simulink library "allblocks_alteradspbuilder2"  (Simulink 7.6)
settings: Solver=ode45  StartTime=0.0  StopTime=10.0  RelTol=1e-3
InitFcn:
  | %% DSPBuilder Start
  | alt_dspbuilder_update_model(bdroot)
  | %% DSPBuilder End
undefined symbols (not defined in the file): alt_dspbuilder_internal_AvalonSTPFC_generate, alt_dspbuilder_internal_init_altlab_flow, alt_dspbuilder_internal_init_blackbox_flow, alt_dspbuilder_internal_initfcn_base_clock, alt_dspbuilder_internal_initfcn_clock, alt_dspbuilder_internal_initfcn_pll, alt_dspbuilder_load_block, alt_dspbuilder_update_external_RAM, Inferred
libraries: allblocks_alteradspbuilder2 x15
(part 1 of 4)
settings Model: ForwardingTableString=||__slOldName__||allblocks_alteradspbuilder2/Stratix III DSP Block||__slNewName__||allblocks_alteradspbuilder2/DSP Block  Creator=swbuild  LastModifiedBy=swbuild

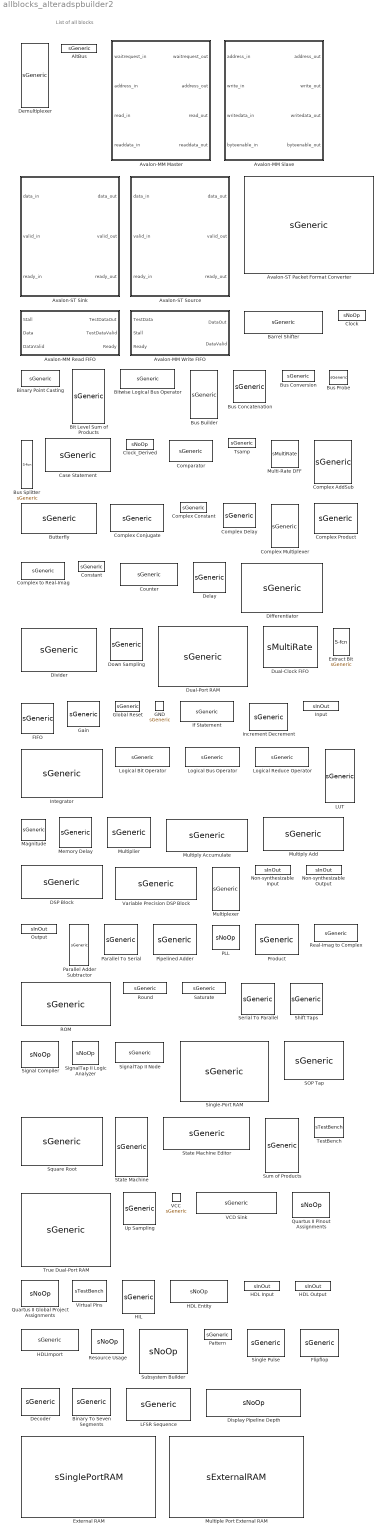
== system allblocks_alteradspbuilder2 ==
  note: List of all blocks
  AltBus : S-Function  LoadFcn=alt_dspbuilder_load_block(gcb, 'BlockFactory', 'com.altera.dspbuilder.blockset.iobus.AltBus');  FunctionName=sGeneric  Parameters=BusType bwl bwr saturate floatingPointInput floatingPointOutput logOutputs logFile  EnableBusSupport=off  mask(AltBus AlteraBlockset){BusType=Signed Integer, bwl=8, bwr=0, saturate=off, floatingPointInput=on, floatingPointOutput=on, logOutputs=off, logFile=D:\\allblocks%5Falteradspbuilder2_AltBus.fixedpointlog}
      mask prompts: BusType "Bus Type"; bwl "[Number Of Bits].[]"; bwr "[].[Number Of Bits]"; saturate "Saturate Output"; floatingPointInput "Allow Floating Point Input For This Block"; floatingPointOutput "Allow Floating Point Output For This Block"
      mask help:
      | Modifies the bus format of a DSP Builder signal. This block can only be used as an internal node in a system, not as an input to or output from the system. If the specified bit width is wider than the input bit width, the bus is sign extended to fit. If it is smaller than the input bit width, you can choose to either truncate or saturate the excess bits
      |
      | If the signal feeding the block has a different format, it is automatically cast to the type specified by the block, and Signal Compiler automatically inserts the hardware cast (if necessary).
      mask init:
      | alt_dspbuilder_init('BlockFactory', 'com.altera.dspbuilder.blockset.iobus.AltBus', { get_param(gcb, 'BusType') bwl bwr saturate floatingPointInput floatingPointOutput logOutputs logFile });
      settings: CopyFcn=alt_dspbuilder_add_block(gcb, 'BlockFactory', 'com.altera.dspbuilder.blockset.iobus.AltBus');  DeleteFcn=com.altera.dspbuilder.simulation.Mask.delete(gcb);  UndoDeleteFcn=alt_dspbuilder_add_block(gcb, 'BlockFactory', 'com.altera.dspbuilder.blockset.iobus.AltBus');  PostSaveFcn=alt_dspbuilder_block_saved(gcb);  NameChangeFcn=alt_dspbuilder_block_renamed(gcb);
      mask Help: helpview(char(com.altera.dspbuilder.simulation.Cache.getBlockTemplate('BlockFactory', 'com.altera.dspbuilder.blockset.iobus.AltBus').getHelpFile))
      mask StyleString: popup(Signed Integer|Unsigned Integer|Signed Fractional|Unsigned Fractional|Single Bit),edit,edit,checkbox,checkbox,checkbox,checkbox,edit
      mask CallbackString: alt_dspbuilder_update_gui('BlockFactory', 'com.altera.dspbuilder.blockset.iobus.AltBus', 'BusType', 0);|||||||
      mask Display:
      | plot([0 0.2 0 1 0.8 1 0], [0 0.5 1 1 0.5 0 0])
      | plot([0.08 0.28 0.08 0.92 0.72 0.92 0.08], [0 0.5 1 1 0.5 0 0])
      | disp('7:0')
  Avalon-MM Master : Subsystem  mask(Avalon-MM Master AlteraBlockset){iofile=D:\\allblocks%5Falteradspbuilder2_Avalon-MM+Master_waitrequest.salt,D:\\allblocks%5Falteradspbuilder2_Avalon-MM+Master_address.capture,D:\\allblocks%5Falteradspbuilder2_Avalon-MM+Master_read.capture,D:\\allblocks%5Falteradspbuilder2_Avalon-MM+Master_readdata.salt,, SpecifyClock=off, clock=, addrWidth=2, addrType=Read, BusType=Signed Integer, bwl=8, bwr=0, byteEnable=off, flowCtrl=off, pipeline=off, flush=off, burst=off, maxBurst=4, irq=off, irq_mode=Prioritized, externalType=Inferred, PORTTYPE=Input}
      mask prompts: SpecifyClock "Specify Clock"; addrWidth "Address Width"; addrType "Address Type"; BusType "DataType"; bwl "[number of bits].[]"; bwr "[].[number of bits]"; byteEnable "Allow Byte Enable"; flowCtrl "Allow Flow Control"; pipeline "Allow Pipeline Transfers"; flush "Use Flush Signal"; burst "Allow Burst Transfers"; maxBurst "Maximum Burst Size"; irq "Receive IRQ"; irq_mode "IRQ Mode"; externalType "External Type"; PORTTYPE "TYPE"
      mask help: Defines a collection of ports for connection to an SOPC Builder system when your design functions as an Avalon Memory-Mapped master interface.
      mask init:
      | alt_dspbuilder_internal_initBusIOBlock('BlockFactory', 'com.altera.dspbuilder.blockset.avalonmm.Master', { iofile get_param(gcb, 'SpecifyClock') clock addrWidth get_param(gcb, 'addrType') get_param(gcb, 'BusType') bwl bwr byteEnable get_param(gcb, 'flowCtrl') get_param(gcb, 'pipeline') get_param(gcb, 'flush') get_param(gcb, 'burst') maxBurst get_param(gcb, 'irq') get_param(gcb, 'irq_mode') externalType PORTTYPE });
      mask Help: helpview(char(com.altera.dspbuilder.simulation.Cache.getBlockTemplate('BlockFactory', 'com.altera.dspbuilder.blockset.avalonmm.Master').getHelpFile))
      mask StyleString: edit,checkbox,edit,edit,popup(Read|Write|Read/Write),popup(Signed Integer|Unsigned Integer|Signed Fractional|Unsigned Fractional),edit,edit,checkbox,checkbox,checkbox,checkbox,checkbox,edit,checkbox,popup(Prioritized|Indiviual Signals),popup(Inferred|Simulink Fixed Point Type|Double),edit
      mask CallbackString: |alt_dspbuilder_update_gui('BlockFactory', 'com.altera.dspbuilder.blockset.avalonmm.Master', 'SpecifyClock', 1);|||alt_dspbuilder_update_gui('BlockFactory', 'com.altera.dspbuilder.blockset.avalonmm.Master', 'addrType', 4);|alt_dspbuilder_update_gui('BlockFactory', 'com.altera.dspbuilder.blockset.avalonmm.Master', 'BusType', 5);||||alt_dspbuilder_update_gui('BlockFactory', 'com.altera.dspbuilder.blockset.avalonmm.Master', 'flowCtrl', 9);|alt_dspbuilder_update_gui('BlockFactory', 'com.altera.dspbuilder.blockset.avalonmm.Master', 'pipeline', 10);|alt_dspbuilder_update_gui('BlockFactory', 'com.altera.dspbuilder.blockset.avalonmm.Master', 'flush', 11);|alt_dspbuilder_update_gui('BlockFactory', 'com.altera.dspbuilder.blockset.avalonmm.Master', 'burst', 12);||alt_dspbuilder_update_gui('BlockFactory', 'com.altera.dspbuilder.blockset.avalonmm.Master', 'irq', 14);|alt_dspbuilder_update_gui('BlockFactory', 'com.altera.dspbuilder.blockset.avalonmm.Master', 'irq_mode', 15);||
      mask Display:
      | plot([-25 15 25 15 -25 -25]*1, [0 0 -10 -20 -20 0] - 0);
      | text(0, -10, 'Wait Request\nibit', 'horizontalAlignment','center','verticalAlignment','middle');
      | plot([-25 15 25 15 -25 -25]*-1, [0 0 -10 -20 -20 0] - 21);
      | plot([11 21 11]*-1, [0 -10 -20] - 21);
      | text(0, -31, 'Address\no1:0', 'horizontalAlignment','center','verticalAlignment','middle');
      | plot([-25 15 25 15 -25 -25]*-1, [0 0 -10 -20 -20 0] - 42);
      | text(0, -52, 'Read\nobit', 'horizontalAlignment','center','verticalAlignment','middle');
      | plot([-25 15 25 15 -25 -25]*1, [0 0 -10 -20 -20 0] - 63);
      | plot([11 21 11]*1, [0 -10 -20] - 63);
      | text(0, -73, 'Read Data\ni7:0', 'horizontalAlignment','center','verticalAlignment','middle');
  Avalon-MM Read FIFO : Subsystem  mask(Avalon-MM Read FIFO AlteraBlockSet){sgn=Signed Integer, bwl=8, bwr=3, depth=11, burst=0}
      mask prompts: sgn "Data Type"; bwl "[number of bits].[]"; bwr "[].[number of bits]"; depth "FIFO Depth"; burst "Max Burst"
      mask help:
      | Avalon-MM Read FIFO
      |
      | Implements a FIFO with Avalon-MM connectivity. Accessed by other Avalon-MM peripherals to obtain datawhen connected in SOPC Builder.
      |
      | Inputs:
      | Stall - Connect to Simulink blocks.
      | 	Used to simulate stall conditions of the Avalon-MM bus.
      | Data - Connect to DSP Builder blocks.
      | 	Used to collect outgoing data from the user design.
      | DataValid - Connect to DSP Builder blocks.
      | 	Should be asserted whenever the signal on the Data port corresponds to real data.
      |
      | Outputs:
      | TestDataOut - Connect to Simulink blocks.
      | 	Corresponds to the data received over the Avalon-MM bus.
      | TestDataValid - Connect to Simulink blocks.
      | 	Asserted whenever TestDataOut corresponds to real data.
      | Ready	- Connect to DSP Builder blocks.
      | 	Used to indicate that the block is ready to receive data.
      mask init:
      | alt_dspbuilder_internal_AvalonFIFO_Init(gcb,1,1, bwl,bwr,depth,burst);
      settings: CopyFcn=set_param(gcbh,'LinkStatus','none');
      mask Help: helpview(fullfile(alt_dspbuilder_get_quartus_rootdir, 'dsp_builder', 'docs', 'AvalonReadFIFO.html'))
      mask StyleString: popup(Signed Integer|Signed Fractional|Unsigned Integer),edit,edit,edit,edit
      mask CallbackString: alt_dspbuilder_internal_AvalonFIFO_Init(gcb,1,0);||||
  Avalon-MM Slave : Subsystem  mask(Avalon-MM Slave AlteraBlockset){iofile=D:\\allblocks%5Falteradspbuilder2_Avalon-MM+Slave_address.salt,D:\\allblocks%5Falteradspbuilder2_Avalon-MM+Slave_write.salt,D:\\allblocks%5Falteradspbuilder2_Avalon-MM+Slave_writedata.salt,D:\\allblocks%5Falteradspbuilder2_Avalon-MM+Slave_byteenable.salt,, SpecifyClock=off, clock=, addrWidth=2, addrAlignment=Dynamic, addrType=Write, BusType=Unsigned Integer, bwl=16, bwr=0, byteEnable=on, flowCtrl=off, pipeline=off, waitStateFormat=Fixed, readWaitStateCycles=0, writeWaitStateCycles=0, readLatencyFormat=Fixed, readLatencyCycles=0, burst=off, maxBurst=4, irq=off, receiveBeginTransfer=off, useChipSelect=off, externalType=Inferred, PORTTYPE=Output}
      mask prompts: SpecifyClock "Specify Clock"; addrWidth "Address Width"; addrAlignment "Address Alignment"; addrType "Address Type"; BusType "DataType"; bwl "[number of bits].[]"; bwr "[].[number of bits]"; byteEnable "Allow Byte Enable"; flowCtrl "Allow Flow Control"; pipeline "Allow Pipeline Transfers"; waitStateFormat "Wait-State Format"; readWaitStateCycles "Read Wait-State Cycles"; writeWaitStateCycles "Write Wait-State Cycles"; readLatencyFormat "Read Latency Format"; readLatencyCycles "Read Latency Cycles"; burst "Allow Burst Transfers"; maxBurst "Maximum Burst Size"; irq "Output IRQ"; receiveBeginTransfer "Receive BeginTransfer"; useChipSelect "Use Chip Select"; externalType "External Type"; PORTTYPE "TYPE"
      mask help: Defines a collection of ports for connection to an SOPC Builder system when your design functions as an Avalon Memory-Mapped slave interface.
      mask init:
      | alt_dspbuilder_internal_initBusIOBlock('BlockFactory', 'com.altera.dspbuilder.blockset.avalonmm.Slave', { iofile get_param(gcb, 'SpecifyClock') clock addrWidth addrAlignment get_param(gcb, 'addrType') get_param(gcb, 'BusType') bwl bwr byteEnable flowCtrl pipeline get_param(gcb, 'waitStateFormat') readWaitStateCycles writeWaitStateCycles readLatencyFormat readLatencyCycles get_param(gcb, 'burst') maxBurst irq receiveBeginTransfer useChipSelect externalType PORTTYPE });
      mask Help: helpview(char(com.altera.dspbuilder.simulation.Cache.getBlockTemplate('BlockFactory', 'com.altera.dspbuilder.blockset.avalonmm.Slave').getHelpFile))
      mask StyleString: edit,checkbox,edit,edit,popup(Dynamic|Native),popup(Read|Write|Read/Write),popup(Signed Integer|Unsigned Integer|Signed Fractional|Unsigned Fractional),edit,edit,checkbox,checkbox,checkbox,popup(Fixed|Variable),edit,edit,popup(Fixed|Variable),edit,checkbox,edit,checkbox,checkbox,checkbox,popup(Inferred|Simulink Fixed Point Type|Double),edit
      mask CallbackString: |alt_dspbuilder_update_gui('BlockFactory', 'com.altera.dspbuilder.blockset.avalonmm.Slave', 'SpecifyClock', 1);||||alt_dspbuilder_update_gui('BlockFactory', 'com.altera.dspbuilder.blockset.avalonmm.Slave', 'addrType', 5);|alt_dspbuilder_update_gui('BlockFactory', 'com.altera.dspbuilder.blockset.avalonmm.Slave', 'BusType', 6);||||||alt_dspbuilder_update_gui('BlockFactory', 'com.altera.dspbuilder.blockset.avalonmm.Slave', 'waitStateFormat', 12);|||||alt_dspbuilder_update_gui('BlockFactory', 'com.altera.dspbuilder.blockset.avalonmm.Slave', 'burst', 17);||||||
      mask Display:
      | plot([-25 15 25 15 -25 -25]*1, [0 0 -10 -20 -20 0] - 0);
      | plot([11 21 11]*1, [0 -10 -20] - 0);
      | text(0, -10, 'Address\ni1:0', 'horizontalAlignment','center','verticalAlignment','middle');
      | plot([-25 15 25 15 -25 -25]*1, [0 0 -10 -20 -20 0] - 21);
      | text(0, -31, 'Write\nibit', 'horizontalAlignment','center','verticalAlignment','middle');
      | plot([-25 15 25 15 -25 -25]*1, [0 0 -10 -20 -20 0] - 42);
      | plot([11 21 11]*1, [0 -10 -20] - 42);
      | text(0, -52, 'Write Data\ni15:0', 'horizontalAlignment','center','verticalAlignment','middle');
      | plot([-25 15 25 15 -25 -25]*1, [0 0 -10 -20 -20 0] - 63);
      | plot([11 21 11]*1, [0 -10 -20] - 63);
      | text(0, -73, 'Byte Enable\ni1:0', 'horizontalAlignment','center','verticalAlignment','middle');
  Avalon-MM Write FIFO : Subsystem  mask(Avalon-MM Write FIFO AlteraBlockSet){sgn=Unsigned Integer, bwl=8, bwr=0, depth=16, burst=8}
      mask prompts: sgn "Data Type"; bwl "[number of bits].[]"; bwr "[].[number of bits]"; depth "FIFO Depth"; burst "Maximum Burst Size"
      mask help:
      | Avalon-MM Write FIFO
      |
      | Implements a FIFO with Avalon-MM connectivity. Used to receive data from other Avalon-MM peripheralswhen connected in SOPC Builder.
      |
      | Inputs:
      | TestData - Connect to Simulink blocks.
      | 	Used to provide simulation data to the Avalon-MM Write FIFO.
      | Stall - Connect to Simulink blocks.
      | 	Used to simulate stall conditions of the Avalon-MM bus.
      | Ready - Connect to DSP Builder blocks.
      | 	Used to indicate that the downstream hardware is ready for data.
      |
      | Outputs:
      | DataOut - Connect to DSP Builder blocks.
      | 	Corresponds to the oldest unsent data sample received on the TestData port.
      | DataValid - Connect to DSP Builder blocks.
      | 	Asserted whenever DataOut corresponds to real data.
      mask init:
      | alt_dspbuilder_internal_AvalonFIFO_Init(gcb,0,1, bwl,bwr,depth,burst);
      settings: CopyFcn=set_param(gcbh,'LinkStatus','none');
      mask Help: helpview(fullfile(alt_dspbuilder_get_quartus_rootdir, 'dsp_builder', 'docs', 'AvalonWriteFifo.html'))
      mask StyleString: popup(Signed Integer|Signed Fractional|Unsigned Integer),edit,edit,edit,edit
      mask CallbackString: alt_dspbuilder_internal_AvalonFIFO_Init(gcb,0,0);||||
  Avalon-ST Packet Format Converter : S-Function  LoadFcn=alt_dspbuilder_load_block(gcb, 'BlockFactory', 'com.altera.dspbuilder.blockset.avalonst.AvalonSTPFC');  InitFcn=alt_dspbuilder_internal_AvalonSTPFC_generate(gcb)  FunctionName=sGeneric  Parameters=NumSinks NumSources splitData multiMapping SymbolWidth userReset SinkFormat1 SinkFormat2 SinkFormat3 SinkFormat4 SinkFormat5 SinkFormat6 SinkFormat7 SinkFormat8 SinkFormat9 SinkFormat10 SinkFormat11 SinkFormat12 SinkFormat13 SinkFormat14 SinkFormat15 SinkFormat16 SymbolsPerBeatSink1 SymbolsPerBeatSink2 SymbolsPerBeatSink3 SymbolsPerBeatSink4 SymbolsPerBeatSink5 SymbolsPerBeatSink6 SymbolsPerBeatSink7 SymbolsPerBeatSink8 SymbolsPerBeatSink9 SymbolsPerBeatSink10 SymbolsPerBeatSink11 SymbolsPerBeatSink12 SymbolsPerBeatSink13 SymbolsPerBeatSink14 SymbolsPerBeatSink15 SymbolsPerBeatSink16 SourceFormat1 SourceFormat2 SourceFormat3 SourceFormat4 SourceFormat5 SourceFormat6 SourceFormat7 SourceFormat8 SourceFormat9 SourceFormat10 SourceFormat11 SourceFormat12 SourceFormat13 SourceFormat14 SourceFormat15 SourceFormat16 SymbolsPerBeatSource1 SymbolsPerBeatSource2 SymbolsPerBeatSource3 SymbolsPerBeatSource4 SymbolsPerBeatSource5 SymbolsPerBeatSource6 SymbolsPerBeatSource7 SymbolsPerBeatSource8 SymbolsPerBeatSource9 SymbolsPerBeatSource10 SymbolsPerBeatSource11 SymbolsPerBeatSource12 SymbolsPerBeatSource13 SymbolsPerBeatSource14 SymbolsPerBeatSource15 SymbolsPerBeatSource16 checksum entityName q_src_files q_src_types inNames inBwls inBwrs inTypes inDelayed outNames outBwls outBwrs outTypes resetNames resetTypes resetLengths id vofile xmlmapfile q_user_lib use_systemC_model n_input_port n_output_port is_megacore array_clocks  EnableBusSupport=off  mask(Avalon Streaming Packet Format Converter){NumSinks=1, NumSources=1, splitData=off, multiMapping=off, SymbolWidth=8, userReset=off, SinkFormat1='Red, Green, Blue', SinkFormat2=, SinkFormat3=, SinkFormat4=, SinkFormat5=, SinkFormat6=, SinkFormat7=, SinkFormat8=, SinkFormat9=, SinkFormat10=, SinkFormat11=, SinkFormat12=, SinkFormat13=, SinkFormat14=, SinkFormat15=, SinkFormat16=, SymbolsPerBeatSink1=1, SymbolsPerBeatSink2=1, SymbolsPerBeatSink3=1, SymbolsPerBeatSink4=1, SymbolsPerBeatSink5=1, SymbolsPerBeatSink6=1, SymbolsPerBeatSink7=1, SymbolsPerBeatSink8=1, SymbolsPerBeatSink9=1, SymbolsPerBeatSink10=1, SymbolsPerBeatSink11=1, SymbolsPerBeatSink12=1, SymbolsPerBeatSink13=1, SymbolsPerBeatSink14=1, SymbolsPerBeatSink15=1, SymbolsPerBeatSink16=1, SourceFormat1='Blue, Green, Red', SourceFormat2=, SourceFormat3=, SourceFormat4=, SourceFormat5=, SourceFormat6=, SourceFormat7=, SourceFormat8=, SourceFormat9=, SourceFormat10=, SourceFormat11=, SourceFormat12=, SourceFormat13=, SourceFormat14=, SourceFormat15=, SourceFormat16=, SymbolsPerBeatSource1=1, SymbolsPerBeatSource2=1, SymbolsPerBeatSource3=1, SymbolsPerBeatSource4=1, SymbolsPerBeatSource5=1, SymbolsPerBeatSource6=1, SymbolsPerBeatSource7=1, SymbolsPerBeatSource8=1, SymbolsPerBeatSource9=1, SymbolsPerBeatSource10=1, SymbolsPerBeatSource11=1, SymbolsPerBeatSource12=1, SymbolsPerBeatSource13=1, SymbolsPerBeatSource14=1, SymbolsPerBeatSource15=1, SymbolsPerBeatSource16=1, checksum=, entityName=, q_src_files=, q_src_types=, inNames=, inBwls=, inBwrs=, inTypes=, inDelayed=, outNames=, outBwls=, outBwrs=, outTypes=, resetNames=, resetTypes=, resetLengths=, id=0, vofile=, xmlmapfile=, q_user_lib=, use_systemC_model=off, n_input_port=0, n_output_port=0, is_megacore=off, array_clocks=}
      mask prompts: NumSinks "Number of Sinks"; NumSources "Number of Sources"; splitData "Split Data"; multiMapping "Multi-Packet Mapping"; SymbolWidth "Symbol Width / bits"; userReset "Use Asynchronous Clear Port (aclr)"; SinkFormat1 "Sink Format 1"; SinkFormat2 "Sink Format 2"; SinkFormat3 "Sink Format 3"; SinkFormat4 "Sink Format 4"; SinkFormat5 "Sink Format 5"; SinkFormat6 "Sink Format 6"; SinkFormat7 "Sink Format 7"; SinkFormat8 "Sink Format 8"; SinkFormat9 "Sink Format 9"; SinkFormat10 "Sink Format 10"; SinkFormat11 "Sink Format 11"; SinkFormat12 "Sink Format 12"; SinkFormat13 "Sink Format 13"; SinkFormat14 "Sink Format 14"; SinkFormat15 "Sink Format 15"; SinkFormat16 "Sink Format 16"; SymbolsPerBeatSink1 "Sink 1 Symbols Per Beat"; SymbolsPerBeatSink2 "Sink 2 Symbols Per Beat"; SymbolsPerBeatSink3 "Sink 3 Symbols Per Beat"; SymbolsPerBeatSink4 "Sink 4 Symbols Per Beat"; SymbolsPerBeatSink5 "Sink 5 Symbols Per Beat"; SymbolsPerBeatSink6 "Sink 6 Symbols Per Beat"; SymbolsPerBeatSink7 "Sink 7 Symbols Per Beat"; SymbolsPerBeatSink8 "Sink 8 Symbols Per Beat"; SymbolsPerBeatSink9 "Sink 9 Symbols Per Beat"; SymbolsPerBeatSink10 "Sink 10 Symbols Per Beat"; SymbolsPerBeatSink11 "Sink 11 Symbols Per Beat"; SymbolsPerBeatSink12 "Sink 12 Symbols Per Beat"; SymbolsPerBeatSink13 "Sink 13 Symbols Per Beat"; SymbolsPerBeatSink14 "Sink 14 Symbols Per Beat"; SymbolsPerBeatSink15 "Sink 15 Symbols Per Beat"; SymbolsPerBeatSink16 "Sink 16 Symbols Per Beat"; SourceFormat1 "Source Format 1"; SourceFormat2 "Source Format 2"; SourceFormat3 "Source Format 3"; SourceFormat4 "Source Format 4"; SourceFormat5 "Source Format 5"; SourceFormat6 "Source Format 6"; SourceFormat7 "Source Format 7"; SourceFormat8 "Source Format 8"; SourceFormat9 "Source Format 9"; SourceFormat10 "Source Format 10"; SourceFormat11 "Source Format 11"; SourceFormat12 "Source Format 12"; SourceFormat13 "Source Format 13"; SourceFormat14 "Source Format 14"; SourceFormat15 "Source Format 15"; SourceFormat16 "Source Format 16"; SymbolsPerBeatSource1 "Source 1 Symbols Per Beat"; SymbolsPerBeatSource2 "Source 2 Symbols Per Beat"; SymbolsPerBeatSource3 "Source 3 Symbols Per Beat"; SymbolsPerBeatSource4 "Source 4 Symbols Per Beat"; SymbolsPerBeatSource5 "Source 5 Symbols Per Beat"; SymbolsPerBeatSource6 "Source 6 Symbols Per Beat"; SymbolsPerBeatSource7 "Source 7 Symbols Per Beat"; SymbolsPerBeatSource8 "Source 8 Symbols Per Beat"; SymbolsPerBeatSource9 "Source 9 Symbols Per Beat"; SymbolsPerBeatSource10 "Source 10 Symbols Per Beat"; SymbolsPerBeatSource11 "Source 11 Symbols Per Beat"; SymbolsPerBeatSource12 "Source 12 Symbols Per Beat"; SymbolsPerBeatSource13 "Source 13 Symbols Per Beat"; SymbolsPerBeatSource14 "Source 14 Symbols Per Beat"; SymbolsPerBeatSource15 "Source 15 Symbols Per Beat"; SymbolsPerBeatSource16 "Source 16 Symbols Per Beat"; is_megacore "n_output_port"
      mask help: Transforms packets received from one block to a different packet format required by another block.
      mask init:
      | alt_dspbuilder_init('BlockFactory', 'com.altera.dspbuilder.blockset.avalonst.AvalonSTPFC', { get_param(gcb, 'NumSinks') get_param(gcb, 'NumSources') splitData multiMapping SymbolWidth userReset SinkFormat1 SinkFormat2 SinkFormat3 SinkFormat4 SinkFormat5 SinkFormat6 SinkFormat7 SinkFormat8 SinkFormat9 SinkFormat10 SinkFormat11 SinkFormat12 SinkFormat13 SinkFormat14 SinkFormat15 SinkFormat16 SymbolsPerBeatSink1 SymbolsPerBeatSink2 SymbolsPerBeatSink3 SymbolsPerBeatSink4 SymbolsPerBeatSink5 SymbolsPerBeatSink6 SymbolsPerBeatSink7 SymbolsPerBeatSink8 SymbolsPerBeatSink9 SymbolsPerBeatSink10 SymbolsPerBeatSink11 SymbolsPerBeatSink12 SymbolsPerBeatSink13 SymbolsPerBeatSink14 SymbolsPerBeatSink15 SymbolsPerBeatSink16 SourceFormat1 SourceFormat2 SourceFormat3 SourceFormat4 SourceFormat5 SourceFormat6 SourceFormat7 SourceFormat8 SourceFormat9 SourceFormat10 SourceFormat11 SourceFormat12 SourceFormat13 SourceFormat14 SourceFormat15 SourceFormat16 SymbolsPerBeatSource1 SymbolsPerBeatSource2 SymbolsPerBeatSource3 SymbolsPerBeatSource4 SymbolsPerBeatSource5 SymbolsPerBeatSource6 SymbolsPerBeatSource7 SymbolsPerBeatSource8 SymbolsPerBeatSource9 SymbolsPerBeatSource10 SymbolsPerBeatSource11 SymbolsPerBeatSource12 SymbolsPerBeatSource13 SymbolsPerBeatSource14 SymbolsPerBeatSource15 SymbolsPerBeatSource16 checksum entityName q_src_files q_src_types inNames inBwls inBwrs inTypes inDelayed outNames outBwls outBwrs outTypes resetNames resetTypes resetLengths id vofile xmlmapfile q_user_lib use_systemC_model n_input_port n_output_port is_megacore array_clocks });
      settings: DeleteFcn=com.altera.dspbuilder.simulation.Mask.delete(gcb);  UndoDeleteFcn=alt_dspbuilder_add_block(gcb, 'BlockFactory', 'com.altera.dspbuilder.blockset.avalonst.AvalonSTPFC');  PostSaveFcn=alt_dspbuilder_block_saved(gcb);  NameChangeFcn=alt_dspbuilder_block_renamed(gcb);
      settings: CopyFcn=|
      | alt_dspbuilder_add_block(gcb, 'BlockFactory', 'com.altera.dspbuilder.blockset.avalonst.AvalonSTPFC');
      | com.altera.dspbuilder.simulation.Mask.simpleInit('BlockFactory', 'com.altera.dspbuilder.blockset.avalonst.AvalonSTPFC', bdroot(gcb), gcb);
      | alt_dspbuilder_internal_init_uniqueidblock(gcb);
      mask Help: helpview(char(com.altera.dspbuilder.simulation.Cache.getBlockTemplate('BlockFactory', 'com.altera.dspbuilder.blockset.avalonst.AvalonSTPFC').getHelpFile))
      mask StyleString: popup(1|2|3|4|5|6|7|8|9|10|11|12|13|14|15|16),popup(1|2|3|4|5|6|7|8|9|10|11|12|13|14|15|16),checkbox,checkbox,edit,checkbox,edit,edit,edit,edit,edit,edit,edit,edit,edit,edit,edit,edit,edit,edit,edit,edit,edit,edit,edit,edit,edit,edit,edit,edit,edit,edit,edit,edit,edit,edit,edit,edit,edit,edit,edit,edit,edit,edit,edit,edit,edit,edit,edit,edit,edit,edit,edit,edit,edit,edit,edit,edit,edit,edit,edit,edit,edit,edit,edit,edit,edit,edit,edit,edit,edit,edit,edit,edit,edit,edit,edit,edit,edit,edit,edit,edit,edit,edit,edit,edit,edit,edit,edit,edit,checkbox,edit,edit,checkbox,edit
      mask CallbackString: alt_dspbuilder_update_gui('BlockFactory', 'com.altera.dspbuilder.blockset.avalonst.AvalonSTPFC', 'NumSinks', 0);|alt_dspbuilder_update_gui('BlockFactory', 'com.altera.dspbuilder.blockset.avalonst.AvalonSTPFC', 'NumSources', 1);|||||||||||||||||||||||||||||||||||||||||||||||||||||||||||||||||||||||||||||||||||||||||||||
      mask TabNameString: General,General,General,General,General,General,Sink Format,Sink Format,Sink Format,Sink Format,Sink Format,Sink Format,Sink Format,Sink Format,Sink Format,Sink Format,Sink Format,Sink Format,Sink Format,Sink Format,Sink Format,Sink Format,Sink Sym/Beat,Sink Sym/Beat,Sink Sym/Beat,Sink Sym/Beat,Sink Sym/Beat,Sink Sym/Beat,Sink Sym/Beat,Sink Sym/Beat,Sink Sym/Beat,Sink Sym/Beat,Sink Sym/Beat,Sink Sym/Beat,Sink Sym/Beat,Sink Sym/Beat,Sink Sym/Beat,Sink Sym/Beat,Source Format,Source Format,Source Format,Source Format,Source Format,Source Format,Source Format,Source Format,Source Format,Source Format,Source Format,Source Format,Source Format,Source Format,Source Format,Source Format,Source Sym/Beat,Source Sym/Beat,Source Sym/Beat,Source Sym/Beat,Source Sym/Beat,Source Sym/Beat,Source Sym/Beat,Source Sym/Beat,Source Sym/Beat,Source Sym/Beat,Source Sym/Beat,Source Sym/Beat,Source Sym/Beat,Source Sym/Beat,Source Sym/Beat,Source Sym/Beat,Source Sym/Beat,Source Sym/Beat,Source Sym/Beat,Source Sym/Beat,Source Sym/Beat,Source Sym/Beat,Source Sym/Beat,Source Sym/Beat,Source Sym/Beat,Source Sym/Beat,Source Sym/Beat,Source Sym/Beat,Source Sym/Beat,Source Sym/Beat,Source Sym/Beat,Source Sym/Beat,Source Sym/Beat,Source Sym/Beat,Source Sym/Beat,Source Sym/Beat,Source Sym/Beat,Source Sym/Beat,Source Sym/Beat,Source Sym/Beat,Source Sym/Beat
      mask Display: disp('Avalon-ST\nPacket Format\nConverter');
  Avalon-ST Sink : Subsystem  mask(Avalon-ST Sink AlteraBlockset){iofile=D:\\allblocks%5Falteradspbuilder2_Avalon-ST+Sink_data.salt,D:\\allblocks%5Falteradspbuilder2_Avalon-ST+Sink_valid.salt,D:\\allblocks%5Falteradspbuilder2_Avalon-ST+Sink_ready.capture,, SpecifyClock=off, clock=, BusType=Unsigned Integer, bwl=8, bwr=0, symbolWidth=8, symbolsPerBeat=1, numOfChannels=0, numOfErrorDescriptors=0, endOfPacket=off, startOfPacket=off, empty=off, readyLatency=1, externalType=Inferred, PORTTYPE=Output}
      mask prompts: SpecifyClock "Specify Clock"; BusType "DataType"; bwl "[number of bits].[]"; bwr "[].[number of bits]"; symbolWidth "Symbol Width"; numOfChannels "Number of Channels"; numOfErrorDescriptors "Number of Error Descriptors"; endOfPacket "Use endofpacket"; startOfPacket "Use startofpacket"; empty "Use empty"; readyLatency "Ready Latency"; externalType "External Type"; PORTTYPE "TYPE"
      mask help: Defines a collection of ports for connection to an SOPC Builder system when your design functions as an Avalon-ST source.
      mask init:
      | alt_dspbuilder_internal_initBusIOBlock('BlockFactory', 'com.altera.dspbuilder.blockset.avalonst.Sink', { iofile get_param(gcb, 'SpecifyClock') clock get_param(gcb, 'BusType') bwl bwr symbolWidth symbolsPerBeat numOfChannels numOfErrorDescriptors endOfPacket startOfPacket empty readyLatency externalType PORTTYPE });
      mask Help: helpview(char(com.altera.dspbuilder.simulation.Cache.getBlockTemplate('BlockFactory', 'com.altera.dspbuilder.blockset.avalonst.Sink').getHelpFile))
      mask StyleString: edit,checkbox,edit,popup(Signed Integer|Unsigned Integer|Signed Fractional|Unsigned Fractional),edit,edit,edit,edit,edit,edit,checkbox,checkbox,checkbox,edit,popup(Inferred|Simulink Fixed Point Type|Double),edit
      mask CallbackString: |alt_dspbuilder_update_gui('BlockFactory', 'com.altera.dspbuilder.blockset.avalonst.Sink', 'SpecifyClock', 1);||alt_dspbuilder_update_gui('BlockFactory', 'com.altera.dspbuilder.blockset.avalonst.Sink', 'BusType', 3);||||||||||||
      mask Display:
      | plot([-25 15 25 15 -25 -25]*1, [0 0 -10 -20 -20 0] - 0);
      | plot([11 21 11]*1, [0 -10 -20] - 0);
      | text(0, -10, 'Data In\ni7:0', 'horizontalAlignment','center','verticalAlignment','middle');
      | plot([-25 15 25 15 -25 -25]*1, [0 0 -10 -20 -20 0] - 21);
      | text(0, -31, 'Valid\nibit', 'horizontalAlignment','center','verticalAlignment','middle');
      | plot([-25 15 25 15 -25 -25]*-1, [0 0 -10 -20 -20 0] - 42);
      | text(0, -52, 'Ready\nobit', 'horizontalAlignment','center','verticalAlignment','middle');
  Avalon-ST Source : Subsystem  mask(Avalon-ST Source AlteraBlockset){iofile=D:\\allblocks%5Falteradspbuilder2_Avalon-ST+Source_data.capture,D:\\allblocks%5Falteradspbuilder2_Avalon-ST+Source_valid.capture,D:\\allblocks%5Falteradspbuilder2_Avalon-ST+Source_ready.salt,, SpecifyClock=off, clock=, BusType=Unsigned Integer, bwl=8, bwr=0, symbolWidth=8, symbolsPerBeat=1, numOfChannels=0, numOfErrorDescriptors=0, endOfPacket=off, startOfPacket=off, empty=off, readyLatency=1, externalType=Inferred, PORTTYPE=Input}
      mask prompts: SpecifyClock "Specify Clock"; BusType "DataType"; bwl "[number of bits].[]"; bwr "[].[number of bits]"; symbolWidth "Symbol Width"; numOfChannels "Number of Channels"; numOfErrorDescriptors "Number of Error Descriptors"; endOfPacket "Use endofpacket"; startOfPacket "Use startofpacket"; empty "Use empty"; readyLatency "Ready Latency"; externalType "External Type"; PORTTYPE "TYPE"
      mask help: Defines a collection of ports for connection to an SOPC Builder system when your design functions as an Avalon-ST source.
      mask init:
      | alt_dspbuilder_internal_initBusIOBlock('BlockFactory', 'com.altera.dspbuilder.blockset.avalonst.Source', { iofile get_param(gcb, 'SpecifyClock') clock get_param(gcb, 'BusType') bwl bwr symbolWidth symbolsPerBeat numOfChannels numOfErrorDescriptors endOfPacket startOfPacket empty readyLatency externalType PORTTYPE });
      mask Help: helpview(char(com.altera.dspbuilder.simulation.Cache.getBlockTemplate('BlockFactory', 'com.altera.dspbuilder.blockset.avalonst.Source').getHelpFile))
      mask StyleString: edit,checkbox,edit,popup(Signed Integer|Unsigned Integer|Signed Fractional|Unsigned Fractional),edit,edit,edit,edit,edit,edit,checkbox,checkbox,checkbox,edit,popup(Inferred|Simulink Fixed Point Type|Double),edit
      mask CallbackString: |alt_dspbuilder_update_gui('BlockFactory', 'com.altera.dspbuilder.blockset.avalonst.Source', 'SpecifyClock', 1);||alt_dspbuilder_update_gui('BlockFactory', 'com.altera.dspbuilder.blockset.avalonst.Source', 'BusType', 3);||||||||||||
      mask Display:
      | plot([-25 15 25 15 -25 -25]*-1, [0 0 -10 -20 -20 0] - 0);
      | plot([11 21 11]*-1, [0 -10 -20] - 0);
      | text(0, -10, 'Data In\no7:0', 'horizontalAlignment','center','verticalAlignment','middle');
      | plot([-25 15 25 15 -25 -25]*-1, [0 0 -10 -20 -20 0] - 21);
      | text(0, -31, 'Valid\nobit', 'horizontalAlignment','center','verticalAlignment','middle');
      | plot([-25 15 25 15 -25 -25]*1, [0 0 -10 -20 -20 0] - 42);
      | text(0, -52, 'Ready\nibit', 'horizontalAlignment','center','verticalAlignment','middle');
  Barrel Shifter : S-Function  LoadFcn=alt_dspbuilder_load_block(gcb, 'BlockFactory', 'com.altera.dspbuilder.blockset.arithmetic.BarrelShifter');  FunctionName=sGeneric  Parameters=BusType bwl bwr pipeline infer_distance distance_length ShiftDirection use_ena use_aclr UseDedicatedCircuitry pipeline_display allowFloatingPointOverride logOutputs logFile  EnableBusSupport=off  mask(BarrelShifter AlteraBlockset){BusType=Signed Integer, bwl=8, bwr=8, pipeline=off, infer_distance=on, distance_length=8, ShiftDirection=Use direction input pin, use_ena=off, use_aclr=off, UseDedicatedCircuitry=off, pipeline_display=0, allowFloatingPointOverride=on, logOutputs=off, logFile=D:\\allblocks%5Falteradspbuilder2_Barrel+Shifter.fixedpointlog}
      mask prompts: BusType "Bus Type"; bwl "[Number Of Bits].[]"; bwr "[].[Number Of Bits]"; pipeline "Enable Pipeline"; infer_distance "Infer size of distance port from input port"; distance_length "Bit width of distance port"; ShiftDirection "Shift Direction"; use_ena "Use Enable Port (ena)"; use_aclr "Use Asynchronous Clear Port (aclr)"; UseDedicatedCircuitry "Use Dedicated Circuitry"; pipeline_display "Number Of Pipeline Stages (Calculated)"; allowFloatingPointOverride "Allow Floating Point Override For This Block"
      mask help:
      | Shifts the input data by the amount set by the distance bus. The Barrel Shifter can shift data to the left (toward the MSB) or to the right (toward the LSB).
      |
      | Inputs:
      |   a : Data input to the barrel shifter
      |   distance : distance to shift
      |   direction : direction to shift
      |
      | Outputs:
      |   r : result after shift such as
      |   r = d << distance when direction = 0 (shift left)
      |   r = d >> distance when direction = 1 (shift right)
      mask init:
      | alt_dspbuilder_init('BlockFactory', 'com.altera.dspbuilder.blockset.arithmetic.BarrelShifter', { get_param(gcb, 'BusType') bwl bwr get_param(gcb, 'pipeline') get_param(gcb, 'infer_distance') distance_length ShiftDirection use_ena use_aclr UseDedicatedCircuitry pipeline_display allowFloatingPointOverride logOutputs logFile });
      settings: CopyFcn=alt_dspbuilder_add_block(gcb, 'BlockFactory', 'com.altera.dspbuilder.blockset.arithmetic.BarrelShifter');  DeleteFcn=com.altera.dspbuilder.simulation.Mask.delete(gcb);  UndoDeleteFcn=alt_dspbuilder_add_block(gcb, 'BlockFactory', 'com.altera.dspbuilder.blockset.arithmetic.BarrelShifter');  PostSaveFcn=alt_dspbuilder_block_saved(gcb);  NameChangeFcn=alt_dspbuilder_block_renamed(gcb);
      mask Help: helpview(char(com.altera.dspbuilder.simulation.Cache.getBlockTemplate('BlockFactory', 'com.altera.dspbuilder.blockset.arithmetic.BarrelShifter').getHelpFile))
      mask StyleString: popup(Signed Integer|Unsigned Integer|Signed Fractional|Unsigned Fractional),edit,edit,checkbox,checkbox,edit,popup(Shift left|Shift right|Use direction input pin),checkbox,checkbox,checkbox,edit,checkbox,checkbox,edit
      mask CallbackString: alt_dspbuilder_update_gui('BlockFactory', 'com.altera.dspbuilder.blockset.arithmetic.BarrelShifter', 'BusType', 0);|||alt_dspbuilder_update_gui('BlockFactory', 'com.altera.dspbuilder.blockset.arithmetic.BarrelShifter', 'pipeline', 3);|alt_dspbuilder_update_gui('BlockFactory', 'com.altera.dspbuilder.blockset.arithmetic.BarrelShifter', 'infer_distance', 4);|||||||||
      mask TabNameString: Main,Main,Main,Main,Main,Main,Optional Ports and Settings,Optional Ports and Settings,Optional Ports and Settings,Optional Ports and Settings,Optional Ports and Settings,Optional Ports and Settings,Optional Ports and Settings,Optional Ports and Settings
      mask Display:
      | port_label('input', 1, 'a(7:0)');
      | port_label('input', 2, 'distance(2:0)');
      | port_label('input', 3, 'direction');
      | port_label('output', 1, 'r(7:0)');
      | 
      | 
      | disp('<<>>');
  Binary Point Casting : S-Function  LoadFcn=alt_dspbuilder_load_block(gcb, 'BlockFactory', 'com.altera.dspbuilder.blockset.iobus.BinaryPointCasting');  FunctionName=sGeneric  Parameters=BusType bwl bwr OutputPointPosition pipeline_display  EnableBusSupport=off  mask(Binary Point Casting AlteraBlockset){BusType=Signed Fractional, bwl=8, bwr=8, OutputPointPosition=6, pipeline_display=0}
      mask prompts: BusType "Bus Type"; bwl "Input [Number Of Bits].[]"; bwr "Input [].[Number Of Bits]"; OutputPointPosition "Output Binary Point Position"; pipeline_display "Number Of Pipeline Stages (Calculated)"
      mask help:
      | Changes the binary point position for a signed fractional bus type, or converts an integer to a fractional bus type.
      | The output bit width remains equal to the input bit width.
      mask init:
      | alt_dspbuilder_init('BlockFactory', 'com.altera.dspbuilder.blockset.iobus.BinaryPointCasting', { get_param(gcb, 'BusType') bwl bwr OutputPointPosition pipeline_display });
      settings: CopyFcn=alt_dspbuilder_add_block(gcb, 'BlockFactory', 'com.altera.dspbuilder.blockset.iobus.BinaryPointCasting');  DeleteFcn=com.altera.dspbuilder.simulation.Mask.delete(gcb);  UndoDeleteFcn=alt_dspbuilder_add_block(gcb, 'BlockFactory', 'com.altera.dspbuilder.blockset.iobus.BinaryPointCasting');  PostSaveFcn=alt_dspbuilder_block_saved(gcb);  NameChangeFcn=alt_dspbuilder_block_renamed(gcb);
      mask Help: helpview(char(com.altera.dspbuilder.simulation.Cache.getBlockTemplate('BlockFactory', 'com.altera.dspbuilder.blockset.iobus.BinaryPointCasting').getHelpFile))
      mask StyleString: popup(Inferred|Signed Integer|Unsigned Integer|Signed Fractional|Unsigned Fractional),edit,edit,edit,edit
      mask CallbackString: alt_dspbuilder_update_gui('BlockFactory', 'com.altera.dspbuilder.blockset.iobus.BinaryPointCasting', 'BusType', 0);||||
      mask Display:
      | port_label('input', 1, '[8]:[8]');
      | port_label('output', 1, '[10][6]');
      | plot([0 0 0.5 0.5 0.5 1 1], [0.5 1 1 0 1 1 0.5])
  Binary To Seven Segments : S-Function  LoadFcn=alt_dspbuilder_load_block(gcb, 'BlockFactory', 'com.altera.dspbuilder.blockset.gatecontrol.BinaryTo7Segment');  FunctionName=sGeneric  Parameters=pipeline_display  EnableBusSupport=off  mask(Binary To Seven Segment AlteraBlockset){pipeline_display=0}
      mask prompts: pipeline_display "Number Of Pipeline Stages (Calculated)"
      mask help:
      | Converts a 4-bit unsigned input bus to a 7-bit output for connection to a seven-segment display.
      |
      | The seven-segment display is set to display the hexadecimal representation of the input number.
      |
      |         Input            Output
      |   Binary  Dec  Hex     Binary  Dec
      |    0000    0    0     1000000   64
      |    0001    1    1     1111001  121
      |    0010    2    2     0100100   36
      |    0011    3    3     0110000   48
      |    0100    4    4     0011001   25
      |    0101    5    5     0010010   18
      |    0110    6    6     0000010    2
      |    0111    7    7     1111000  120
      |    1000    8    8     0000000    0
      |    1001    9    9     0010000   16
      |    1010   10    A     0001000    8
      |    1011   11    b     0000011    3
      |    1100   12    C     1000110   70
      |    1101   13    d     1000001   33
      |    1110   14    E     0000110    6
      |    1111   15    F     0001110   14
      mask init:
      | alt_dspbuilder_init('BlockFactory', 'com.altera.dspbuilder.blockset.gatecontrol.BinaryTo7Segment', { pipeline_display });
      settings: CopyFcn=alt_dspbuilder_add_block(gcb, 'BlockFactory', 'com.altera.dspbuilder.blockset.gatecontrol.BinaryTo7Segment');  DeleteFcn=com.altera.dspbuilder.simulation.Mask.delete(gcb);  UndoDeleteFcn=alt_dspbuilder_add_block(gcb, 'BlockFactory', 'com.altera.dspbuilder.blockset.gatecontrol.BinaryTo7Segment');  PostSaveFcn=alt_dspbuilder_block_saved(gcb);  NameChangeFcn=alt_dspbuilder_block_renamed(gcb);
      mask Help: helpview(char(com.altera.dspbuilder.simulation.Cache.getBlockTemplate('BlockFactory', 'com.altera.dspbuilder.blockset.gatecontrol.BinaryTo7Segment').getHelpFile))
      mask Display:
      | port_label('input', 1, '(3:0)');
      | port_label('output', 1, '(6:0)');
  Bit Level Sum of Products : S-Function  LoadFcn=alt_dspbuilder_load_block(gcb, 'BlockFactory', 'com.altera.dspbuilder.blockset.arithmetic.BitSumProducts');  FunctionName=sGeneric  Parameters=number_of_coefficients BusType bwl bwr coefficients register_inputs pipeline_display use_ena use_sclr allowFloatingPointOverride logOutputs logFile  EnableBusSupport=off  mask(BitSumProducts AlteraBlockset){number_of_coefficients=4, BusType=Signed Integer, bwl=8, bwr=0, coefficients=[1 2 3 4 5 6 7 8], register_inputs=on, pipeline_display=1, use_ena=off, use_sclr=off, allowFloatingPointOverride=on, logOutputs=off, logFile=D:\\allblocks%5Falteradspbuilder2_Bit+Level+Sum+of+Products.fixedpointlog}
      mask prompts: number_of_coefficients "Number of Coefficients (1-8)"; BusType "Bus Type"; bwl "Coefficient Number Of Bits"; bwr "[].[Number Of Bits]"; coefficients "Signed Integer Fixed-Coefficient Values (Ci)"; register_inputs "Register Inputs"; pipeline_display "Number Of Pipeline Stages (Calculated)"; use_ena "Use Enable Port (ena)"; use_sclr "Use Synchronous Clear Port (sclr)"; allowFloatingPointOverride "Allow Floating Point Override For This Block"
      mask help:
      | Performs a sum of the multiplication of one-bit inputs by signed integer fixed coefficients:
      |
      | q = a(0)C0 + ... + a(i)Ci + ... + a(n-1)Cn-1
      |
      |    q     : Output result
      |    a(i)  : One-bit input data
      |    Ci    : Signed integer fixed coefficient
      |    n     : Number of coefficients, range [1,8]
      mask init:
      | alt_dspbuilder_init('BlockFactory', 'com.altera.dspbuilder.blockset.arithmetic.BitSumProducts', { number_of_coefficients BusType bwl bwr coefficients get_param(gcb, 'register_inputs') pipeline_display use_ena use_sclr allowFloatingPointOverride logOutputs logFile });
      settings: CopyFcn=alt_dspbuilder_add_block(gcb, 'BlockFactory', 'com.altera.dspbuilder.blockset.arithmetic.BitSumProducts');  DeleteFcn=com.altera.dspbuilder.simulation.Mask.delete(gcb);  UndoDeleteFcn=alt_dspbuilder_add_block(gcb, 'BlockFactory', 'com.altera.dspbuilder.blockset.arithmetic.BitSumProducts');  PostSaveFcn=alt_dspbuilder_block_saved(gcb);  NameChangeFcn=alt_dspbuilder_block_renamed(gcb);
      mask Help: helpview(char(com.altera.dspbuilder.simulation.Cache.getBlockTemplate('BlockFactory', 'com.altera.dspbuilder.blockset.arithmetic.BitSumProducts').getHelpFile))
      mask StyleString: edit,popup(Signed Integer|Unsigned Integer|Signed Fractional|Unsigned Fractional),edit,edit,edit,checkbox,edit,checkbox,checkbox,checkbox,checkbox,edit
      mask CallbackString: |||||alt_dspbuilder_update_gui('BlockFactory', 'com.altera.dspbuilder.blockset.arithmetic.BitSumProducts', 'register_inputs', 5);||||||
      mask TabNameString: Main,Main,Main,Main,Main,Main,Main,Optional Ports,Optional Ports,Optional Ports,Optional Ports,Optional Ports
      mask Display:
      | port_label('input', 1, 'a0');
      | port_label('input', 2, 'a1');
      | port_label('input', 3, 'a2');
      | port_label('input', 4, 'a3');
      | port_label('output', 1, 'q(9:0)');
      | plot([0.9 0.75 0.85 0.75 0.9], [0.15 0.15 0.1 0.05 0.05])
  Bitwise Logical Bus Operator : S-Function  LoadFcn=alt_dspbuilder_load_block(gcb, 'BlockFactory', 'com.altera.dspbuilder.blockset.gatecontrol.BitwiseLogicalBus');  FunctionName=sGeneric  Parameters=BusType bwl bwr LogicalOperator pipeline_display  EnableBusSupport=off  mask(Bitwise Logical Bus Operator AlteraBlockset){BusType=Signed Integer, bwl=8, bwr=0, LogicalOperator=AND, pipeline_display=0}
      mask prompts: BusType "Bus Type"; bwl "[Number Of Bits].[]"; bwr "[].[Number Of Bits]"; LogicalOperator "Logical Operation"; pipeline_display "Number Of Pipeline Stages (Calculated)"
      mask help: Performs bitwise-AND, bitwise-exclusive-OR, or bitwise-inclusive-OR logical operations on two input buses.
      mask init:
      | alt_dspbuilder_init('BlockFactory', 'com.altera.dspbuilder.blockset.gatecontrol.BitwiseLogicalBus', { get_param(gcb, 'BusType') bwl bwr get_param(gcb, 'LogicalOperator') pipeline_display });
      settings: CopyFcn=alt_dspbuilder_add_block(gcb, 'BlockFactory', 'com.altera.dspbuilder.blockset.gatecontrol.BitwiseLogicalBus');  DeleteFcn=com.altera.dspbuilder.simulation.Mask.delete(gcb);  UndoDeleteFcn=alt_dspbuilder_add_block(gcb, 'BlockFactory', 'com.altera.dspbuilder.blockset.gatecontrol.BitwiseLogicalBus');  PostSaveFcn=alt_dspbuilder_block_saved(gcb);  NameChangeFcn=alt_dspbuilder_block_renamed(gcb);
      mask Help: helpview(char(com.altera.dspbuilder.simulation.Cache.getBlockTemplate('BlockFactory', 'com.altera.dspbuilder.blockset.gatecontrol.BitwiseLogicalBus').getHelpFile))
      mask StyleString: popup(Inferred|Signed Integer|Unsigned Integer|Signed Fractional|Unsigned Fractional),edit,edit,popup(AND|OR|XOR),edit
      mask CallbackString: alt_dspbuilder_update_gui('BlockFactory', 'com.altera.dspbuilder.blockset.gatecontrol.BitwiseLogicalBus', 'BusType', 0);|||alt_dspbuilder_update_gui('BlockFactory', 'com.altera.dspbuilder.blockset.gatecontrol.BitwiseLogicalBus', 'LogicalOperator', 3);|
      mask Display:
      | port_label('input', 1, 'a(7:0)');
      | port_label('input', 2, 'b(7:0)');
      | port_label('output', 1, 'q(7:0)');
      | plot([-exp((pi/2:.1:1.5*pi)*i) -1+i -1-i 0-i])
      | 
      | 
      | 
      | 
      | 
      | disp('AND')
  Bus Builder : S-Function  LoadFcn=alt_dspbuilder_load_block(gcb, 'BlockFactory', 'com.altera.dspbuilder.blockset.iobus.BusBuilder');  FunctionName=sGeneric  Parameters=BusType bwl bwr pipeline_display  EnableBusSupport=off  mask(BusBuilder AlteraBlockset){BusType=Signed Integer, bwl=8, bwr=1, pipeline_display=0}
      mask prompts: BusType "Bus Type"; bwl "[Number Of Bits].[]"; bwr "[].[Number Of Bits]"; pipeline_display "Number Of Pipeline Stages (Calculated)"
      mask help: Constructs an output bus from single-bit inputs. The output bus can be signed integer, unsigned integer or signed binary fractional format. You can specify the number of bits in each case.
      mask init:
      | alt_dspbuilder_init('BlockFactory', 'com.altera.dspbuilder.blockset.iobus.BusBuilder', { get_param(gcb, 'BusType') bwl bwr pipeline_display });
      settings: CopyFcn=alt_dspbuilder_add_block(gcb, 'BlockFactory', 'com.altera.dspbuilder.blockset.iobus.BusBuilder');  DeleteFcn=com.altera.dspbuilder.simulation.Mask.delete(gcb);  UndoDeleteFcn=alt_dspbuilder_add_block(gcb, 'BlockFactory', 'com.altera.dspbuilder.blockset.iobus.BusBuilder');  PostSaveFcn=alt_dspbuilder_block_saved(gcb);  NameChangeFcn=alt_dspbuilder_block_renamed(gcb);
      mask Help: helpview(char(com.altera.dspbuilder.simulation.Cache.getBlockTemplate('BlockFactory', 'com.altera.dspbuilder.blockset.iobus.BusBuilder').getHelpFile))
      mask StyleString: popup(Signed Integer|Unsigned Integer|Signed Fractional|Unsigned Fractional),edit,edit,edit
      mask CallbackString: alt_dspbuilder_update_gui('BlockFactory', 'com.altera.dspbuilder.blockset.iobus.BusBuilder', 'BusType', 0);|||
      mask Display:
      | port_label('input', 1, '0');
      | port_label('input', 2, '1');
      | port_label('input', 3, '2');
      | port_label('input', 4, '3');
      | port_label('input', 5, '4');
      | port_label('input', 6, '5');
      | port_label('input', 7, '6');
      | port_label('input', 8, '7');
      | port_label('output', 1, '(7:0)');
      | plot([0 0.75 0.75 1], [1 1 0.6 0.6])
      | plot([0 0.75 0.75 1], [0 0 0.4 0.4])
  Bus Concatenation : S-Function  LoadFcn=alt_dspbuilder_load_block(gcb, 'BlockFactory', 'com.altera.dspbuilder.blockset.iobus.BusConcatenate');  FunctionName=sGeneric  Parameters=isSigned awidth bwidth pipeline_display  EnableBusSupport=off  mask(Bus Concatenate AlteraBlockset){isSigned=off, awidth=8, bwidth=1, pipeline_display=0}
      mask prompts: isSigned "Output is Signed"; awidth "Width Of Input a"; bwidth "Width Of Input b"; pipeline_display "Number Of Pipeline Stages (Calculated)"
      mask help:
      | Concatenates two buses.
      |
      | The block has two inputs, a and b. These may be signed integer or unsigned integer. The output width is width(a) + width(b).
      | Input a becomes the MSB part of the output, input b becomes the LSB part.
      mask init:
      | alt_dspbuilder_init('BlockFactory', 'com.altera.dspbuilder.blockset.iobus.BusConcatenate', { isSigned awidth bwidth pipeline_display });
      settings: CopyFcn=alt_dspbuilder_add_block(gcb, 'BlockFactory', 'com.altera.dspbuilder.blockset.iobus.BusConcatenate');  DeleteFcn=com.altera.dspbuilder.simulation.Mask.delete(gcb);  UndoDeleteFcn=alt_dspbuilder_add_block(gcb, 'BlockFactory', 'com.altera.dspbuilder.blockset.iobus.BusConcatenate');  PostSaveFcn=alt_dspbuilder_block_saved(gcb);  NameChangeFcn=alt_dspbuilder_block_renamed(gcb);
      mask Help: helpview(char(com.altera.dspbuilder.simulation.Cache.getBlockTemplate('BlockFactory', 'com.altera.dspbuilder.blockset.iobus.BusConcatenate').getHelpFile))
      mask Display:
      | port_label('input', 1, 'a(7:0)');
      | port_label('input', 2, 'b(0:0)');
      | port_label('output', 1, 'ab(8:0)');
      | plot([0 0.75 0.75 1], [1 1 0.6 0.6])
      | plot([0 0.75 0.75 1], [0 0 0.4 0.4])
  Bus Conversion : S-Function  LoadFcn=alt_dspbuilder_load_block(gcb, 'BlockFactory', 'com.altera.dspbuilder.blockset.iobus.BusConversion');  FunctionName=sGeneric  Parameters=BusType ibwl ibwr bwl bwr bitToConnectToOutputLSB round saturate pipeline_display  EnableBusSupport=off  mask(Bus Conversion AlteraBlockset){BusType=Signed Integer, ibwl=8, ibwr=1, bwl=4, bwr=1, bitToConnectToOutputLSB=3, round=off, saturate=off, pipeline_display=0}
      mask prompts: BusType "Bus Type"; ibwl "Input [Number Of Bits].[]"; ibwr "Input [].[Number Of Bits]"; bwl "Output [Number Of Bits].[]"; bwr "Output [].[Number Of Bits]"; bitToConnectToOutputLSB "Input Bit Connected To Output LSB"; pipeline_display "Number Of Pipeline Stages (Calculated)"
      mask help:
      | Extracts a subsection of a bus including bus type and width conversion.
      |
      | If the input is in signed binary fractional format, you should specify a left bit width (number of integer bits) and a right bit width (number of fractional bits) for the output bus. If the input is an integer, you should instead specify which input bit to connect to the output LSB.
      |
      | If Input Bit Connected To Output LSB is on, the input bit indexing starts from 0. This option cannot be used with signed fractional type or in conjunction with rounding.
      mask init:
      | alt_dspbuilder_init('BlockFactory', 'com.altera.dspbuilder.blockset.iobus.BusConversion', { get_param(gcb, 'BusType') ibwl ibwr bwl bwr bitToConnectToOutputLSB get_param(gcb, 'round') saturate pipeline_display });
      settings: CopyFcn=alt_dspbuilder_add_block(gcb, 'BlockFactory', 'com.altera.dspbuilder.blockset.iobus.BusConversion');  DeleteFcn=com.altera.dspbuilder.simulation.Mask.delete(gcb);  UndoDeleteFcn=alt_dspbuilder_add_block(gcb, 'BlockFactory', 'com.altera.dspbuilder.blockset.iobus.BusConversion');  PostSaveFcn=alt_dspbuilder_block_saved(gcb);  NameChangeFcn=alt_dspbuilder_block_renamed(gcb);
      mask Help: helpview(char(com.altera.dspbuilder.simulation.Cache.getBlockTemplate('BlockFactory', 'com.altera.dspbuilder.blockset.iobus.BusConversion').getHelpFile))
      mask StyleString: popup(Signed Integer|Unsigned Integer|Signed Fractional|Unsigned Fractional),edit,edit,edit,edit,edit,checkbox,checkbox,edit
      mask CallbackString: alt_dspbuilder_update_gui('BlockFactory', 'com.altera.dspbuilder.blockset.iobus.BusConversion', 'BusType', 0);||||||alt_dspbuilder_update_gui('BlockFactory', 'com.altera.dspbuilder.blockset.iobus.BusConversion', 'round', 6);||
      mask Display:
      | port_label('input', 1, '(7:0)');
      | port_label('output', 1, '(6:3)');
      | plot([0 0 0.5 0.5 1 1], [0.5 0 0 1 1 0.5])
  Bus Probe : S-Function  LoadFcn=alt_dspbuilder_load_block(gcb, 'BlockFactory', 'com.altera.dspbuilder.blockset.altlab.BusProbe');  InitFcn=alt_dspbuilder_internal_init_altlab_flow;  FunctionName=sGeneric  Parameters=display max_value min_value max_bits  EnableBusSupport=off  mask(BusProbe AlteraBlockset){display=Maximum number of integer bits required during simulation, max_value=nan, min_value=nan, max_bits=0}
      mask prompts: display "Display in Symbol"; max_value "Maximum value reached during simulation"; min_value "Minimum value reached during simulation"; max_bits "Maximum number of integer bits required during simulation"
      mask help:
      | The Bus Probe (BP) block is a sink block, which can be placed on any node of the model.
      |
      | The BP block does not have any hardware representation and therefore does not appear in the VHDL RTL representation generated by the SignalCompiler block.
      |
      | The Display in Symbol parameter selects the graphical shape of the symbol in your model and the information that is reported on the symbol:
      |  - Circle shape : Maximum number of integer bits required during simulation
      |  - Rectangle shape : Maximum or minimum value reached during simulation
      |
      | After simulating the model, the BP block back-annotates the following information in its edit box:
      |  - Maximum value reached during simulation
      |  - Minimum value reached during simulation
      |  - Maximum number of integer bits required during simulation
      mask init:
      | alt_dspbuilder_init('BlockFactory', 'com.altera.dspbuilder.blockset.altlab.BusProbe', { display max_value min_value max_bits });
      settings: CopyFcn=alt_dspbuilder_add_block(gcb, 'BlockFactory', 'com.altera.dspbuilder.blockset.altlab.BusProbe');  DeleteFcn=com.altera.dspbuilder.simulation.Mask.delete(gcb);  UndoDeleteFcn=alt_dspbuilder_add_block(gcb, 'BlockFactory', 'com.altera.dspbuilder.blockset.altlab.BusProbe');  PostSaveFcn=alt_dspbuilder_block_saved(gcb);  NameChangeFcn=alt_dspbuilder_block_renamed(gcb);
      mask Help: helpview(char(com.altera.dspbuilder.simulation.Cache.getBlockTemplate('BlockFactory', 'com.altera.dspbuilder.blockset.altlab.BusProbe').getHelpFile))
      mask StyleString: popup(Maximum number of integer bits required during simulation|Maximum value reached during simulation|Minimum value reached during simulation),edit,edit,edit
      mask Display:
      | plot([-exp((0:.1:2.5*pi)*i) -i])
      | disp(max_bits)
  Bus Splitter : S-Function  LoadFcn=alt_dspbuilder_load_block(gcb, 'BlockFactory', 'com.altera.dspbuilder.blockset.iobus.BusSplitter');  FunctionName=sGeneric  Parameters=BusType bwl bwr pipeline_display  EnableBusSupport=off  mask(Bus Splitter AlteraBlockset){BusType=Signed Integer, bwl=8, bwr=0, pipeline_display=0}
      mask prompts: BusType "Bus Type"; bwl "[Number Of Bits].[]"; bwr "[].[Number Of Bits]"; pipeline_display "Number Of Pipeline Stages (Calculated)"
      mask help:
      | Splits a bus into single-bit outputs.
      |
      | The output ports are numbered from least significant to most significant bit. You can choose the bus type that you wish to use, and specify the number of bits on either side of the binary point.
      mask init:
      | alt_dspbuilder_init('BlockFactory', 'com.altera.dspbuilder.blockset.iobus.BusSplitter', { get_param(gcb, 'BusType') bwl bwr pipeline_display });
      settings: CopyFcn=alt_dspbuilder_add_block(gcb, 'BlockFactory', 'com.altera.dspbuilder.blockset.iobus.BusSplitter');  DeleteFcn=com.altera.dspbuilder.simulation.Mask.delete(gcb);  UndoDeleteFcn=alt_dspbuilder_add_block(gcb, 'BlockFactory', 'com.altera.dspbuilder.blockset.iobus.BusSplitter');  PostSaveFcn=alt_dspbuilder_block_saved(gcb);  NameChangeFcn=alt_dspbuilder_block_renamed(gcb);
      mask Help: helpview(char(com.altera.dspbuilder.simulation.Cache.getBlockTemplate('BlockFactory', 'com.altera.dspbuilder.blockset.iobus.BusSplitter').getHelpFile))
      mask StyleString: popup(Signed Integer|Unsigned Integer|Signed Fractional|Unsigned Fractional),edit,edit,edit
      mask CallbackString: alt_dspbuilder_update_gui('BlockFactory', 'com.altera.dspbuilder.blockset.iobus.BusSplitter', 'BusType', 0);|||
      mask Display:
      | port_label('input', 1, '(7:0)');
      | port_label('output', 1, '0');
      | port_label('output', 2, '1');
      | port_label('output', 3, '2');
      | port_label('output', 4, '3');
      | port_label('output', 5, '4');
      | port_label('output', 6, '5');
      | port_label('output', 7, '6');
      | port_label('output', 8, '7');
      | plot([0 0.75 0.75 1], [0.6 0.6 1 1])
      | plot([0 0.75 0.75 1], [0.4 0.4 0 0])
  Butterfly : S-Function  LoadFcn=alt_dspbuilder_load_block(gcb, 'BlockFactory', 'com.altera.dspbuilder.blockset.complex.Butterfly');  FunctionName=sGeneric  Parameters=BusType ibwl ibwr pipeline pipeline_display full_resolution obwl obwr olsb constant_W W_real W_imag dedicated_circuitry use_ena use_aclr allowFloatingPointOverride logOutputs logFile  EnableBusSupport=off  mask(Butterfly Complex AlteraBlockset){BusType=Signed Integer, ibwl=8, ibwr=8, pipeline=6, pipeline_display=6, full_resolution=on, obwl=18, obwr=8, olsb=3, constant_W=off, W_real=1, W_imag=1, dedicated_circuitry=Auto, use_ena=off, use_aclr=off, allowFloatingPointOverride=on, logOutputs=off, logFile=D:\\allblocks%5Falteradspbuilder2_Butterfly%3A%3AA.fixedpointlog,D:\\allblocks%5Falteradspbuilder2_Butterfly%3A%3AB.fixedpointlog,}
      mask prompts: BusType "Bus Type"; ibwl "Input Bit Width (a,b,W)"; ibwr "Input [].[Number Of Bits]"; pipeline "Number Of Pipeline Stages (>= 3)"; pipeline_display "Number Of Pipeline Stages (Calculated)"; full_resolution "Full Resolution for Output Type"; obwl "Output Bit Width (A,B)"; obwr "Output [].[Number Of Bits]"; olsb "Output Truncated LSB"; constant_W "W is Constant"; W_real "W (real)"; W_imag "W (imaginary)"; dedicated_circuitry "Dedicated Multiplier Circuitry"; use_ena "Use Enable Port (ena)"; use_aclr "Use Asynchronous Clear Port (aclr)"; allowFloatingPointOverride "Allow Floating Point Override For This Block"
      mask help:
      | Performs the following arithmetic operation on complex signed integer numbers:
      |  A = a + b*W
      |  B = a - b*W
      |
      | Turn off "Full Resolution for Output Result" to truncate output. "Output Number of Bits" then specifies the width of the output, and "Output Truncated LSB" the number of least-significant bits to be dropped.
      mask init:
      | alt_dspbuilder_init('BlockFactory', 'com.altera.dspbuilder.blockset.complex.Butterfly', { get_param(gcb, 'BusType') ibwl ibwr pipeline pipeline_display get_param(gcb, 'full_resolution') obwl obwr olsb get_param(gcb, 'constant_W') W_real W_imag dedicated_circuitry use_ena use_aclr allowFloatingPointOverride logOutputs logFile });
      settings: CopyFcn=alt_dspbuilder_add_block(gcb, 'BlockFactory', 'com.altera.dspbuilder.blockset.complex.Butterfly');  DeleteFcn=com.altera.dspbuilder.simulation.Mask.delete(gcb);  UndoDeleteFcn=alt_dspbuilder_add_block(gcb, 'BlockFactory', 'com.altera.dspbuilder.blockset.complex.Butterfly');  PostSaveFcn=alt_dspbuilder_block_saved(gcb);  NameChangeFcn=alt_dspbuilder_block_renamed(gcb);
      mask Help: helpview(char(com.altera.dspbuilder.simulation.Cache.getBlockTemplate('BlockFactory', 'com.altera.dspbuilder.blockset.complex.Butterfly').getHelpFile))
      mask StyleString: popup(Signed Integer|Unsigned Integer|Signed Fractional|Unsigned Fractional),edit,edit,edit,edit,checkbox,edit,edit,edit,checkbox,edit,edit,popup(Auto|Yes|No),checkbox,checkbox,checkbox,checkbox,edit
      mask CallbackString: alt_dspbuilder_update_gui('BlockFactory', 'com.altera.dspbuilder.blockset.complex.Butterfly', 'BusType', 0);|||||alt_dspbuilder_update_gui('BlockFactory', 'com.altera.dspbuilder.blockset.complex.Butterfly', 'full_resolution', 5);||||alt_dspbuilder_update_gui('BlockFactory', 'com.altera.dspbuilder.blockset.complex.Butterfly', 'constant_W', 9);||||||||
      mask TabNameString: Main,Main,Main,Main,Main,Optional Port Sizing,Optional Port Sizing,Optional Port Sizing,Optional Port Sizing,Optional Ports and Settings,Optional Ports and Settings,Optional Ports and Settings,Optional Ports and Settings,Optional Ports and Settings,Optional Ports and Settings,Optional Ports and Settings,Optional Ports and Settings,Optional Ports and Settings
      mask Display:
      | port_label('input', 1, 'a(7:0)');
      | port_label('input', 2, 'b(7:0)');
      | port_label('input', 3, 'W(7:0)');
      | port_label('output', 1, 'A(17:0)');
      | port_label('output', 2, 'B(17:0)');
      | plot([0 0.14 0.43 0.57 0.86 1 0.86 0.57 0.57 0.86 1 0.86 0.57 0.43 0.43 0.43 0.14 0], [1 1 0.75 0.75 1 1 1 0.75 0.5 0.25 0.25 0.25 0.5 0.5 0.75 0.5 0.25 0.25])
  Case Statement : S-Function  LoadFcn=alt_dspbuilder_load_block(gcb, 'BlockFactory', 'com.altera.dspbuilder.blockset.gatecontrol.Case');  FunctionName=sGeneric  Parameters=numOutputs case_expression formatted_case_expression BusType bwl bwr pipeline pipeline_display hasDefault  EnableBusSupport=off  mask(Case Statement AlteraBlockset){numOutputs=4, case_expression=1|2|3,4,5|-1,7, formatted_case_expression=00000001|00000010|00000011,00000100,00000101|11111111,00000111, BusType=Signed Integer, bwl=8, bwr=0, pipeline=off, pipeline_display=0, hasDefault=off}
      mask prompts: case_expression "Case Statement"; BusType "Data Bus Type"; bwl "[Number Of Bits].[]"; bwr "[].[Number Of Bits]"; pipeline "Enable Pipeline"; pipeline_display "Number Of Pipeline Stages (Calculated)"; hasDefault "Provide Default Case"
      mask help:
      | Compares an input signal (which must be signed or unsigned integer) with a set of values (or cases). A single-bit output is generated for each case. You can implement multiple cases using a comma (,) to separate each case. A comma at the end of the case values is ignored.
      | You can have multiple conditions for each case by using a pipe (|) to separate the conditions. For example, for four cases with the first of which having two conditions, you would enter 1|2,3,4,5 in the Case Values box.
      mask init:
      | alt_dspbuilder_init('BlockFactory', 'com.altera.dspbuilder.blockset.gatecontrol.Case', { numOutputs case_expression formatted_case_expression get_param(gcb, 'BusType') bwl bwr pipeline pipeline_display hasDefault });
      settings: CopyFcn=alt_dspbuilder_add_block(gcb, 'BlockFactory', 'com.altera.dspbuilder.blockset.gatecontrol.Case');  DeleteFcn=com.altera.dspbuilder.simulation.Mask.delete(gcb);  UndoDeleteFcn=alt_dspbuilder_add_block(gcb, 'BlockFactory', 'com.altera.dspbuilder.blockset.gatecontrol.Case');  PostSaveFcn=alt_dspbuilder_block_saved(gcb);  NameChangeFcn=alt_dspbuilder_block_renamed(gcb);
      mask Help: helpview(char(com.altera.dspbuilder.simulation.Cache.getBlockTemplate('BlockFactory', 'com.altera.dspbuilder.blockset.gatecontrol.Case').getHelpFile))
      mask StyleString: edit,edit,edit,popup(Signed Integer|Unsigned Integer),edit,edit,checkbox,edit,checkbox
      mask CallbackString: |||alt_dspbuilder_update_gui('BlockFactory', 'com.altera.dspbuilder.blockset.gatecontrol.Case', 'BusType', 3);|||||
      mask Display:
      | port_label('output', 1, '1 | 2 | 3');
      | port_label('output', 2, '4');
      | port_label('output', 3, '5 | -1');
      | port_label('output', 4, '7');
      | disp('case')
  Clock : S-Function  LoadFcn=|  InitFcn=alt_dspbuilder_internal_initfcn_base_clock(gcb);  FunctionName=sNoOp  Parameters=ClockPeriod ClockPeriodUnit SampleTime ResetLatency ResetRegisterCascadeDepth SimulationStartCycle PhaseOffset Reset ResetType Export  EnableBusSupport=off  mask(BaseClock AlteraBlockset){ClockPeriod=20, ClockPeriodUnit=ns, SampleTime=1, ResetLatency=0, ResetRegisterCascadeDepth=0, SimulationStartCycle=5, PhaseOffset=0, Reset=aclr, ResetType=Active Low, Export=off}
      | alt_dspbuilder_load_block(gcb, 'BlockFactory', 'com.altera.dspbuilder.blockset.altlab.BaseClock');
      | alt_dspbuilder_load_clock(gcb, 'BlockFactory', 'com.altera.dspbuilder.blockset.altlab.BaseClock');
      mask prompts: ClockPeriod "Real-World Clock Period"; ClockPeriodUnit "Period Unit"; SampleTime "Simulink Sample Time"; ResetLatency "Latency on reset signal due to any added synchronized reset handling"; ResetRegisterCascadeDepth "Extra registers needed for reset synchronization"; SimulationStartCycle "Cycle testbench simulation should start"; PhaseOffset "Phase offset (cycle)"; Reset "Reset Name"; ResetType "Reset Type"; Export "Export As Output Pin"
      mask help:
      | Used in the top level of a design to set the base hardware clock domain.
      |
      | The block name is used as the name of the clock signal and must be a valid VHDL identifier.
      |
      | There can be zero or one base clock in a design and an error is issued if you try to use more than one base clock. You can choose the required units and enter any positive value using the specified units. However, the clock period must be greater than 1ps but less than 2.1ms.
      |
      | If no base clock exists in the design, a default clock (clock) with a 20ns real-world period and a Simulink sample time of 1 is automatically created along with a default Active Low reset (aclr).
      |
      | Additional clocks can be derived from the base clock by adding a Clock_Derived block.
      |
      | Note: Each clock must have a unique reset name. As all clock blocks have the same default reset name (aclr) you must take care to specify a valid unique name when using multiple clocks.
      mask init:
      | alt_dspbuilder_init('BlockFactory', 'com.altera.dspbuilder.blockset.altlab.BaseClock', { ClockPeriod ClockPeriodUnit SampleTime ResetLatency ResetRegisterCascadeDepth SimulationStartCycle PhaseOffset Reset ResetType Export });
      settings: CopyFcn=alt_dspbuilder_add_block(gcb, 'BlockFactory', 'com.altera.dspbuilder.blockset.altlab.BaseClock');  DeleteFcn=com.altera.dspbuilder.simulation.Mask.delete(gcb);  UndoDeleteFcn=alt_dspbuilder_add_block(gcb, 'BlockFactory', 'com.altera.dspbuilder.blockset.altlab.BaseClock');  PostSaveFcn=alt_dspbuilder_block_saved(gcb);  NameChangeFcn=alt_dspbuilder_block_renamed(gcb);
      mask Help: helpview(char(com.altera.dspbuilder.simulation.Cache.getBlockTemplate('BlockFactory', 'com.altera.dspbuilder.blockset.altlab.BaseClock').getHelpFile))
      mask StyleString: edit,popup(ps|ns|us|ms|sec),edit,edit,edit,edit,popup(0|1/2|1/4|1/8|1/16|1/32),edit,popup(Active Low|Active High|Synchronized Active Low|Synchronized Active High),checkbox
      mask Display:
      | plot([0 0.375 0.375 0.5 0.5 0.625 0.625 0.75 0.75 1 1 0 0], [0 0 0.17 0.17 0 0 0.17 0.17 0 0 1 1 0])
      | plot([0.08 0.08 1 1], [0 1 1 0])
      | disp('20 ns');
  Clock_Derived : S-Function  LoadFcn=|  InitFcn=alt_dspbuilder_internal_initfcn_clock(gcb);  FunctionName=sNoOp  Parameters=ClockNumerator ClockDenominator ResetLatency ResetRegisterCascadeDepth SimulationStartCycle PhaseOffset Reset ResetType Export  EnableBusSupport=off  mask(Clock AlteraBlockset){ClockNumerator=2, ClockDenominator=1, ResetLatency=0, ResetRegisterCascadeDepth=0, SimulationStartCycle=5, PhaseOffset=0, Reset=aclr, ResetType=Active Low, Export=off}
      | alt_dspbuilder_load_block(gcb, 'BlockFactory', 'com.altera.dspbuilder.blockset.altlab.Clock');
      | alt_dspbuilder_load_clock(gcb, 'BlockFactory', 'com.altera.dspbuilder.blockset.altlab.Clock');
      mask prompts: ClockNumerator "Base Clock Multiplicand Numerator"; ClockDenominator "Base Clock Multiplicand Denominator"; ResetLatency "Latency on reset signal due to any added synchronized reset handling"; ResetRegisterCascadeDepth "Extra registers needed for reset synchronization"; SimulationStartCycle "Cycle testbench simulation should start"; PhaseOffset "Phase offset (cycle)"; Reset "Reset Name"; ResetType "Reset Type"; Export "Export As Output Pin"
      mask help:
      | The Clock_Derived block can be used in the top level of your design to add additional clock pins to your design. These clocks must be specified as a rational multiple of the base clock for simulation purposes.
      |
      | The block name is used as the name of the clock signal and must be a valid VHDL identifier.
      |
      | You can specify the numerator and denominator multiplicands used to calculate the derived clock. However, the resulting clock period should be greater than 1ps but less than 2.1ms.
      |
      | If no base clock is set, in the design, a 20ns base clock is automatically created and used to determine the derived clock period. You must use a Clock block to set the base clock if you want the sample time to be anything other than 1.
      |
      | Note:   Each clock must have a unique reset name. As all clock blocks have the same default reset name (aclr) you must take care to specify a valid unique name when using multiple clocks.
      mask init:
      | alt_dspbuilder_init('BlockFactory', 'com.altera.dspbuilder.blockset.altlab.Clock', { ClockNumerator ClockDenominator ResetLatency ResetRegisterCascadeDepth SimulationStartCycle PhaseOffset Reset ResetType Export });
      settings: CopyFcn=alt_dspbuilder_add_block(gcb, 'BlockFactory', 'com.altera.dspbuilder.blockset.altlab.Clock');  DeleteFcn=com.altera.dspbuilder.simulation.Mask.delete(gcb);  UndoDeleteFcn=alt_dspbuilder_add_block(gcb, 'BlockFactory', 'com.altera.dspbuilder.blockset.altlab.Clock');  PostSaveFcn=alt_dspbuilder_block_saved(gcb);  NameChangeFcn=alt_dspbuilder_block_renamed(gcb);
      mask Help: helpview(char(com.altera.dspbuilder.simulation.Cache.getBlockTemplate('BlockFactory', 'com.altera.dspbuilder.blockset.altlab.Clock').getHelpFile))
      mask StyleString: edit,edit,edit,edit,edit,popup(0|1/2|1/4|1/8|1/16|1/32),edit,popup(Active Low|Active High|Synchronized Active Low|Synchronized Active High),checkbox
      mask Display:
      | plot([0 0.375 0.375 0.5 0.5 0.625 0.625 0.75 0.75 1 1 0 0], [0 0 0.17 0.17 0 0 0.17 0.17 0 0 1 1 0])
      | disp('x2/1');
  Comparator : S-Function  LoadFcn=alt_dspbuilder_load_block(gcb, 'BlockFactory', 'com.altera.dspbuilder.blockset.arithmetic.Comparator');  FunctionName=sGeneric  Parameters=direction pipeline_display allowFloatingPointOverride logOutputs logFile  EnableBusSupport=off  mask(Comparator AlteraBlockset){direction=a == b, pipeline_display=0, allowFloatingPointOverride=on, logOutputs=off, logFile=D:\\allblocks%5Falteradspbuilder2_Comparator.fixedpointlog}
      mask prompts: direction "Operator"; pipeline_display "Number Of Pipeline Stages (Calculated)"; allowFloatingPointOverride "Allow Floating Point Override For This Block"
      mask help:
      | Compares two Simulink signals and returns a single bit.
      |
      | The Comparator block implicitly understands the input data type (for example, signed binary or unsigned integer) and produces a single-bit output.
      mask init:
      | alt_dspbuilder_init('BlockFactory', 'com.altera.dspbuilder.blockset.arithmetic.Comparator', { get_param(gcb, 'direction') pipeline_display allowFloatingPointOverride logOutputs logFile });
      settings: CopyFcn=alt_dspbuilder_add_block(gcb, 'BlockFactory', 'com.altera.dspbuilder.blockset.arithmetic.Comparator');  DeleteFcn=com.altera.dspbuilder.simulation.Mask.delete(gcb);  UndoDeleteFcn=alt_dspbuilder_add_block(gcb, 'BlockFactory', 'com.altera.dspbuilder.blockset.arithmetic.Comparator');  PostSaveFcn=alt_dspbuilder_block_saved(gcb);  NameChangeFcn=alt_dspbuilder_block_renamed(gcb);
      mask Help: helpview(char(com.altera.dspbuilder.simulation.Cache.getBlockTemplate('BlockFactory', 'com.altera.dspbuilder.blockset.arithmetic.Comparator').getHelpFile))
      mask StyleString: popup(a == b|a ~= b|a < b|a <= b|a >= b|a > b),edit,checkbox,checkbox,edit
      mask CallbackString: alt_dspbuilder_update_gui('BlockFactory', 'com.altera.dspbuilder.blockset.arithmetic.Comparator', 'direction', 0);||||
      mask Display:
      | port_label('input', 1, 'a');
      | port_label('input', 2, 'b');
      | disp('==');
  Complex AddSub : S-Function  LoadFcn=alt_dspbuilder_load_block(gcb, 'BlockFactory', 'com.altera.dspbuilder.blockset.complex.AddSub');  FunctionName=sGeneric  Parameters=number_of_inputs direction use_pipeline pipeline_display phase_selection use_ena use_aclr allowFloatingPointOverride logOutputs logFile  EnableBusSupport=off  mask(AddSub Complex AlteraBlockset){number_of_inputs=2, direction=+, use_pipeline=on, pipeline_display=1, phase_selection=1, use_ena=off, use_aclr=off, allowFloatingPointOverride=on, logOutputs=off, logFile=D:\\allblocks%5Falteradspbuilder2_Complex+AddSub.fixedpointlog}
      mask prompts: number_of_inputs "Number Of Inputs"; direction "Add (+) Sub (-)"; use_pipeline "Enable Pipeline (Variable Length)"; pipeline_display "Number Of Pipeline Stages (Calculated)"; phase_selection "Clock Phase Selection"; use_ena "Use Enable Port (ena)"; use_aclr "Use Asynchronous Clear Port (aclr)"; allowFloatingPointOverride "Allow Floating Point Override For This Block"
      mask help: Performs addition or subtraction on a specified number of scalar complex inputs.
      mask init:
      | alt_dspbuilder_init('BlockFactory', 'com.altera.dspbuilder.blockset.complex.AddSub', { number_of_inputs direction get_param(gcb, 'use_pipeline') pipeline_display phase_selection use_ena use_aclr allowFloatingPointOverride logOutputs logFile });
      settings: CopyFcn=alt_dspbuilder_add_block(gcb, 'BlockFactory', 'com.altera.dspbuilder.blockset.complex.AddSub');  DeleteFcn=com.altera.dspbuilder.simulation.Mask.delete(gcb);  UndoDeleteFcn=alt_dspbuilder_add_block(gcb, 'BlockFactory', 'com.altera.dspbuilder.blockset.complex.AddSub');  PostSaveFcn=alt_dspbuilder_block_saved(gcb);  NameChangeFcn=alt_dspbuilder_block_renamed(gcb);
      mask Help: helpview(char(com.altera.dspbuilder.simulation.Cache.getBlockTemplate('BlockFactory', 'com.altera.dspbuilder.blockset.complex.AddSub').getHelpFile))
      mask CallbackString: ||alt_dspbuilder_update_gui('BlockFactory', 'com.altera.dspbuilder.blockset.complex.AddSub', 'use_pipeline', 2);|||||||
      mask TabNameString: Main,Main,Main,Main,Optional Ports,Optional Ports,Optional Ports,Optional Ports,Optional Ports,Optional Ports
      mask Display:
      | port_label('input', 1, '+');
      | port_label('input', 2, '+');
      | port_label('output', 1, 'R');
      | plot([-i +i -exp((pi/2:.02*pi:1.5*pi)*i)])
      | disp('+');
  Complex Conjugate : S-Function  LoadFcn=alt_dspbuilder_load_block(gcb, 'BlockFactory', 'com.altera.dspbuilder.blockset.complex.Conjugate');  FunctionName=sGeneric  Parameters=operation register_inputs pipeline_display use_ena use_aclr allowFloatingPointOverride logOutputs logFile  EnableBusSupport=off  mask(Conjugate Complex AlteraBlockset){operation=Conjugate, register_inputs=off, pipeline_display=0, use_ena=off, use_aclr=off, allowFloatingPointOverride=on, logOutputs=off, logFile=D:\\allblocks%5Falteradspbuilder2_Complex+Conjugate.fixedpointlog}
      mask prompts: register_inputs "Register Inputs"; pipeline_display "Number Of Pipeline Stages (Calculated)"; use_ena "Use Enable Port (ena)"; use_aclr "Use Asynchronous Clear Port (aclr)"; allowFloatingPointOverride "Allow Floating Point Override For This Block"
      mask help:
      | Outputs a fixed-point complex conjugate value by performing simple arithmetic operations on the complex inputs.
      |
      | The operation can optionally be conjugate, negative or negative conjugate.
      | For an input w = x +iy, the block returns:
      |
      |  - Conjugate : x - iy
      |  - Negative : -x - iy
      |  - Negative Conjugate : -x + iy
      mask init:
      | alt_dspbuilder_init('BlockFactory', 'com.altera.dspbuilder.blockset.complex.Conjugate', { operation get_param(gcb, 'register_inputs') pipeline_display use_ena use_aclr allowFloatingPointOverride logOutputs logFile });
      settings: CopyFcn=alt_dspbuilder_add_block(gcb, 'BlockFactory', 'com.altera.dspbuilder.blockset.complex.Conjugate');  DeleteFcn=com.altera.dspbuilder.simulation.Mask.delete(gcb);  UndoDeleteFcn=alt_dspbuilder_add_block(gcb, 'BlockFactory', 'com.altera.dspbuilder.blockset.complex.Conjugate');  PostSaveFcn=alt_dspbuilder_block_saved(gcb);  NameChangeFcn=alt_dspbuilder_block_renamed(gcb);
      mask Help: helpview(char(com.altera.dspbuilder.simulation.Cache.getBlockTemplate('BlockFactory', 'com.altera.dspbuilder.blockset.complex.Conjugate').getHelpFile))
      mask StyleString: popup(Conjugate|Negative|Negative Conjugate),checkbox,edit,checkbox,checkbox,checkbox,checkbox,edit
      mask CallbackString: |alt_dspbuilder_update_gui('BlockFactory', 'com.altera.dspbuilder.blockset.complex.Conjugate', 'register_inputs', 1);||||||
      mask TabNameString: Main,Main,Main,Optional Ports,Optional Ports,Optional Ports,Optional Ports,Optional Ports
      mask Display:
      | port_label('input', 1, 'w');
      | port_label('output', 1, 'c');
      | disp('x - iy');
  Complex Constant : S-Function  LoadFcn=alt_dspbuilder_load_block(gcb, 'BlockFactory', 'com.altera.dspbuilder.blockset.complex.Constant');  FunctionName=sGeneric  Parameters=mask_cst_real mask_cst_imag BusType bwl bwr allowFloatingPointOverride logOutputs logFile SpecifyClock  EnableBusSupport=off  mask(Constant Complex AlteraBlockset){mask_cst_real=5, mask_cst_imag=5, BusType=Signed Integer, bwl=8, bwr=0, allowFloatingPointOverride=on, logOutputs=off, logFile=D:\\allblocks%5Falteradspbuilder2_Complex+Constant.fixedpointlog, SpecifyClock=off, clock=}
      mask prompts: mask_cst_real "Real Part"; mask_cst_imag "Imaginary Part"; BusType "Bus Type"; bwl "[Number Of Bits].[]"; bwr "[].[Number Of Bits]"; allowFloatingPointOverride "Allow Floating Point Override For This Block"; SpecifyClock "Specify Clock"
      mask help: Outputs a fixed-point complex constant value.
      mask init:
      | alt_dspbuilder_init('BlockFactory', 'com.altera.dspbuilder.blockset.complex.Constant', { mask_cst_real mask_cst_imag get_param(gcb, 'BusType') bwl bwr allowFloatingPointOverride logOutputs logFile get_param(gcb, 'SpecifyClock') clock });
      settings: CopyFcn=alt_dspbuilder_add_block(gcb, 'BlockFactory', 'com.altera.dspbuilder.blockset.complex.Constant');  DeleteFcn=com.altera.dspbuilder.simulation.Mask.delete(gcb);  UndoDeleteFcn=alt_dspbuilder_add_block(gcb, 'BlockFactory', 'com.altera.dspbuilder.blockset.complex.Constant');  PostSaveFcn=alt_dspbuilder_block_saved(gcb);  NameChangeFcn=alt_dspbuilder_block_renamed(gcb);
      mask Help: helpview(char(com.altera.dspbuilder.simulation.Cache.getBlockTemplate('BlockFactory', 'com.altera.dspbuilder.blockset.complex.Constant').getHelpFile))
      mask StyleString: edit,edit,popup(Signed Integer|Unsigned Integer|Signed Fractional|Unsigned Fractional),edit,edit,checkbox,checkbox,edit,checkbox,edit
      mask CallbackString: ||alt_dspbuilder_update_gui('BlockFactory', 'com.altera.dspbuilder.blockset.complex.Constant', 'BusType', 2);||||||alt_dspbuilder_update_gui('BlockFactory', 'com.altera.dspbuilder.blockset.complex.Constant', 'SpecifyClock', 8);|
      mask Display:
      | plot([0 0.8 1 0.8 0  0 0.72 0.92 0.72], [0 0  0.5 1 1 0 0 0.5 1]);
      | disp(5 + 5i);
  Complex Delay : S-Function  LoadFcn=alt_dspbuilder_load_block(gcb, 'BlockFactory', 'com.altera.dspbuilder.blockset.complex.Delay');  FunctionName=sGeneric  Parameters=pipeline pipeline_display ClockPhase use_ena use_sclr allowFloatingPointOverride logOutputs logFile  EnableBusSupport=off  mask(Delay Complex AlteraBlockset){pipeline=1, pipeline_display=1, ClockPhase=1, use_ena=off, use_sclr=off, allowFloatingPointOverride=on, logOutputs=off, logFile=D:\\allblocks%5Falteradspbuilder2_Complex+Delay.fixedpointlog}
      mask prompts: pipeline "Number Of Pipeline Stages"; pipeline_display "Number Of Pipeline Stages (Calculated)"; ClockPhase "Clock Phase Selection"; use_ena "Use Enable Port (ena)"; use_sclr "Use Synchronous Clear port (sclr)"; allowFloatingPointOverride "Allow Floating Point Override For This Block"
      mask help:
      | delays the incoming data by an amount specified by the Number of Pipeline Stages parameter. The input must be a complex number.
      |
      | The Number of Pipeline levels specifies the delay length of the block and must be greater than or equal to 1.
      |
      | The Clock Phase Selection is a binary string which sets the phases in which the block is enabled.
      | For example, 0100 means the delay block is enabled only on the second phase of four.
      mask init:
      | alt_dspbuilder_init('BlockFactory', 'com.altera.dspbuilder.blockset.complex.Delay', { pipeline pipeline_display ClockPhase use_ena use_sclr allowFloatingPointOverride logOutputs logFile });
      settings: CopyFcn=alt_dspbuilder_add_block(gcb, 'BlockFactory', 'com.altera.dspbuilder.blockset.complex.Delay');  DeleteFcn=com.altera.dspbuilder.simulation.Mask.delete(gcb);  UndoDeleteFcn=alt_dspbuilder_add_block(gcb, 'BlockFactory', 'com.altera.dspbuilder.blockset.complex.Delay');  PostSaveFcn=alt_dspbuilder_block_saved(gcb);  NameChangeFcn=alt_dspbuilder_block_renamed(gcb);
      mask Help: helpview(char(com.altera.dspbuilder.simulation.Cache.getBlockTemplate('BlockFactory', 'com.altera.dspbuilder.blockset.complex.Delay').getHelpFile))
      mask TabNameString: Main,Main,Optional Ports and Settings,Optional Ports and Settings,Optional Ports and Settings,Optional Ports and Settings,Optional Ports and Settings,Optional Ports and Settings
      mask Display:
      | port_label('input', 1, 'd');
      | port_label('output', 1, 'q');
      | disp('z^{-1}','texmode','on');
  Complex Multiplexer : S-Function  LoadFcn=alt_dspbuilder_load_block(gcb, 'BlockFactory', 'com.altera.dspbuilder.blockset.complex.Multiplexer');  FunctionName=sGeneric  Parameters=numInputs pipeline oneHot pipeline_display allowFloatingPointOverride logOutputs logFile use_ena use_aclr  EnableBusSupport=off  mask(Multiplexer Complex AlteraBlockset){numInputs=6, pipeline=0, oneHot=off, pipeline_display=0, allowFloatingPointOverride=on, logOutputs=off, logFile=D:\\allblocks%5Falteradspbuilder2_Complex+Multiplexer.fixedpointlog, use_ena=off, use_aclr=off}
      mask prompts: numInputs "Number of Input Data Lines"; pipeline "Number of Pipeline Stages"; oneHot "One Hot Select Bus"; pipeline_display "Number Of Pipeline Stages (Calculated)"; allowFloatingPointOverride "Allow Floating Point Override For This Block"; use_ena "Use Enable Port (ena)"; use_aclr "Use Asynchronous Clear Port (aclr)"
      mask help: Multiplexes N complex inputs to one complex output. The select port sel is a non-complex scalar
      mask init:
      | alt_dspbuilder_init('BlockFactory', 'com.altera.dspbuilder.blockset.complex.Multiplexer', { numInputs pipeline oneHot pipeline_display allowFloatingPointOverride logOutputs logFile use_ena use_aclr });
      settings: CopyFcn=alt_dspbuilder_add_block(gcb, 'BlockFactory', 'com.altera.dspbuilder.blockset.complex.Multiplexer');  DeleteFcn=com.altera.dspbuilder.simulation.Mask.delete(gcb);  UndoDeleteFcn=alt_dspbuilder_add_block(gcb, 'BlockFactory', 'com.altera.dspbuilder.blockset.complex.Multiplexer');  PostSaveFcn=alt_dspbuilder_block_saved(gcb);  NameChangeFcn=alt_dspbuilder_block_renamed(gcb);
      mask Help: helpview(char(com.altera.dspbuilder.simulation.Cache.getBlockTemplate('BlockFactory', 'com.altera.dspbuilder.blockset.complex.Multiplexer').getHelpFile))
      mask TabNameString: Main,Main,Main,Main,Main,Main,Main,Optional Ports,Optional Ports
      mask Display:
      | port_label('input', 1, 'sel(2:0)');
      | port_label('input', 2, '0-');
      | port_label('input', 3, '1-');
      | port_label('input', 4, '2-');
      | port_label('input', 5, '3-');
      | port_label('input', 6, '4-');
      | port_label('input', 7, '5-');
      | plot([0 0 0.25 1 1 0.25 0], [0 1 1 0.875 0.125 0 0])
      | disp('MUX');
  Complex Product : S-Function  LoadFcn=alt_dspbuilder_load_block(gcb, 'BlockFactory', 'com.altera.dspbuilder.blockset.complex.Product');  FunctionName=sGeneric  Parameters=BusType bwl bwr pipeline_register pipeline_display use_ena use_aclr UseDedicatedCircuitry allowFloatingPointOverride logOutputs logFile  EnableBusSupport=off  mask(Product Complex AlteraBlockset){BusType=Inferred, bwl=8, bwr=0, pipeline_register=Inputs Multiplier and Adder, pipeline_display=3, use_ena=off, use_aclr=off, UseDedicatedCircuitry=off, allowFloatingPointOverride=on, logOutputs=off, logFile=D:\\allblocks%5Falteradspbuilder2_Complex+Product.fixedpointlog}
      mask prompts: BusType "Bus Type"; bwl "Input [Number Of Bits].[]"; bwr "Input [].[Number Of Bits]"; pipeline_register "Pipeline Register"; pipeline_display "Number Of Pipeline Stages (Calculated)"; use_ena "Use Enable Port (ena)"; use_aclr "Use Asynchronous Clear Port (aclr)"; UseDedicatedCircuitry "Use Dedicated Circuitry"; allowFloatingPointOverride "Allow Floating Point Override For This Block"
      mask help:
      | Performs output multiplication of two scalar complex inputs. Operand a is multiplied by operand b and the result output on r as shown by the following equation:
      |  r = a x b
      mask init:
      | alt_dspbuilder_init('BlockFactory', 'com.altera.dspbuilder.blockset.complex.Product', { get_param(gcb, 'BusType') bwl bwr pipeline_register pipeline_display use_ena use_aclr UseDedicatedCircuitry allowFloatingPointOverride logOutputs logFile });
      settings: CopyFcn=alt_dspbuilder_add_block(gcb, 'BlockFactory', 'com.altera.dspbuilder.blockset.complex.Product');  DeleteFcn=com.altera.dspbuilder.simulation.Mask.delete(gcb);  UndoDeleteFcn=alt_dspbuilder_add_block(gcb, 'BlockFactory', 'com.altera.dspbuilder.blockset.complex.Product');  PostSaveFcn=alt_dspbuilder_block_saved(gcb);  NameChangeFcn=alt_dspbuilder_block_renamed(gcb);
      mask Help: helpview(char(com.altera.dspbuilder.simulation.Cache.getBlockTemplate('BlockFactory', 'com.altera.dspbuilder.blockset.complex.Product').getHelpFile))
      mask StyleString: popup(Inferred|Signed Integer|Unsigned Integer|Signed Fractional|Unsigned Fractional),edit,edit,popup(No Register|Inputs Only|Multiplier Only|Adder Only|Inputs and Multiplier|Inputs and Adder|Multiplier and Adder|Inputs Multiplier and Adder),edit,checkbox,checkbox,checkbox,checkbox,checkbox,edit
      mask CallbackString: alt_dspbuilder_update_gui('BlockFactory', 'com.altera.dspbuilder.blockset.complex.Product', 'BusType', 0);||||||||||
      mask TabNameString: Main,Main,Main,Main,Main,Optional Ports,Optional Ports,Optional Ports,Optional Ports,Optional Ports,Optional Ports
      mask Display:
      | port_label('input', 1, 'a');
      | port_label('input', 2, 'b');
      | port_label('output', 1, 'r   ');
      | plot([0 0 0 1 0], [0 1 0 0.5 1])
      | disp('X  ');
  Complex to Real-Imag : S-Function  LoadFcn=alt_dspbuilder_load_block(gcb, 'BlockFactory', 'com.altera.dspbuilder.blockset.complex.ComplexToRealImag');  FunctionName=sGeneric  Parameters=BusType bwl bwr pipeline_display allowFloatingPointOverride logOutputs logFile  EnableBusSupport=off  mask(ComplexToRealImag AlteraBlockset){BusType=Signed Integer, bwl=8, bwr=0, pipeline_display=0, allowFloatingPointOverride=on, logOutputs=off, logFile=D:\\allblocks%5Falteradspbuilder2_Complex+to+Real-Imag%3A%3Aoutput%5Freal.fixedpointlog,D:\\allblocks%5Falteradspbuilder2_Complex+to+Real-Imag%3A%3Aoutput%5Fimag.fixedpointlog,}
      mask prompts: BusType "Bus Type"; bwl "[Number Of Bits].[]"; bwr "[].[Number Of Bits]"; pipeline_display "Number Of Pipeline Stages (Calculated)"; allowFloatingPointOverride "Allow Floating Point Override For This Block"
      mask help: Constructs a fixed-point real and fixed-point imaginary output from a complex input.
      mask init:
      | alt_dspbuilder_init('BlockFactory', 'com.altera.dspbuilder.blockset.complex.ComplexToRealImag', { get_param(gcb, 'BusType') bwl bwr pipeline_display allowFloatingPointOverride logOutputs logFile });
      settings: CopyFcn=alt_dspbuilder_add_block(gcb, 'BlockFactory', 'com.altera.dspbuilder.blockset.complex.ComplexToRealImag');  DeleteFcn=com.altera.dspbuilder.simulation.Mask.delete(gcb);  UndoDeleteFcn=alt_dspbuilder_add_block(gcb, 'BlockFactory', 'com.altera.dspbuilder.blockset.complex.ComplexToRealImag');  PostSaveFcn=alt_dspbuilder_block_saved(gcb);  NameChangeFcn=alt_dspbuilder_block_renamed(gcb);
      mask Help: helpview(char(com.altera.dspbuilder.simulation.Cache.getBlockTemplate('BlockFactory', 'com.altera.dspbuilder.blockset.complex.ComplexToRealImag').getHelpFile))
      mask StyleString: popup(Signed Integer|Unsigned Integer|Signed Fractional|Unsigned Fractional),edit,edit,edit,checkbox,checkbox,edit
      mask CallbackString: alt_dspbuilder_update_gui('BlockFactory', 'com.altera.dspbuilder.blockset.complex.ComplexToRealImag', 'BusType', 0);||||||
      mask Display:
      | port_label('input', 1, 'c (7:0)');
      | port_label('output', 1, 'r (7:0)');
      | port_label('output', 2, 'i (7:0)');
  Constant : S-Function  LoadFcn=alt_dspbuilder_load_block(gcb, 'BlockFactory', 'com.altera.dspbuilder.blockset.iobus.Constant');  FunctionName=sGeneric  Parameters=mask_cst BusType bwl bwr roundMode satMode SpecifyClock allowFloatingPointOverride logOutputs logFile  EnableBusSupport=off  mask(Constant AlteraBlockset){mask_cst=5, BusType=Signed Integer, bwl=8, bwr=0, roundMode=Truncate, satMode=Wrap, SpecifyClock=off, clock=, allowFloatingPointOverride=on, logOutputs=off, logFile=D:\\allblocks%5Falteradspbuilder2_Constant.fixedpointlog}
      mask prompts: mask_cst "Constant Value"; BusType "Bus Type"; bwl "[Number Of Bits].[]"; bwr "[].[Number Of Bits]"; roundMode "Rounding Mode"; satMode "Saturation Mode"; SpecifyClock "Specify Clock"; allowFloatingPointOverride "Allow Floating Point Override For This Block"
      mask help: Specifies a constant bus. The options available depend on the selected bus type.
      mask init:
      | alt_dspbuilder_init('BlockFactory', 'com.altera.dspbuilder.blockset.iobus.Constant', { mask_cst get_param(gcb, 'BusType') bwl bwr roundMode satMode get_param(gcb, 'SpecifyClock') clock allowFloatingPointOverride logOutputs logFile });
      settings: CopyFcn=alt_dspbuilder_add_block(gcb, 'BlockFactory', 'com.altera.dspbuilder.blockset.iobus.Constant');  DeleteFcn=com.altera.dspbuilder.simulation.Mask.delete(gcb);  UndoDeleteFcn=alt_dspbuilder_add_block(gcb, 'BlockFactory', 'com.altera.dspbuilder.blockset.iobus.Constant');  PostSaveFcn=alt_dspbuilder_block_saved(gcb);  NameChangeFcn=alt_dspbuilder_block_renamed(gcb);
      mask Help: helpview(char(com.altera.dspbuilder.simulation.Cache.getBlockTemplate('BlockFactory', 'com.altera.dspbuilder.blockset.iobus.Constant').getHelpFile))
      mask StyleString: edit,popup(Signed Integer|Unsigned Integer|Signed Fractional|Unsigned Fractional|Single Bit),edit,edit,popup(Truncate|Round Towards Zero|Round Away From Zero|Round To Plus Infinity|Convergent Rounding),popup(Wrap|Saturate),checkbox,edit,checkbox,checkbox,edit
      mask CallbackString: |alt_dspbuilder_update_gui('BlockFactory', 'com.altera.dspbuilder.blockset.iobus.Constant', 'BusType', 1);|||||alt_dspbuilder_update_gui('BlockFactory', 'com.altera.dspbuilder.blockset.iobus.Constant', 'SpecifyClock', 6);||||
      mask Display:
      | plot([0 40 50 40 0  0 36 46 36], [0 0  10 20 20 0 0 10 20]);
      | disp(5);
  Counter : S-Function  LoadFcn=alt_dspbuilder_load_block(gcb, 'BlockFactory', 'com.altera.dspbuilder.blockset.arithmetic.Counter');  FunctionName=sGeneric  Parameters=BusType bwl bwr use_modulo modulo SpecifyClock direction use_sload use_sset svalue use_clk_ena use_ena use_sclr pipeline_display  EnableBusSupport=off  mask(Counter AlteraBlockset){BusType=Signed Integer, bwl=8, bwr=0, use_modulo=on, modulo=255, SpecifyClock=off, clock=, direction=Increment, use_sload=off, use_sset=off, svalue=1, use_clk_ena=off, use_ena=off, use_sclr=off, pipeline_display=1}
      mask prompts: BusType "Bus Type"; bwl "[Number Of Bits].[]"; bwr "[].[Number Of Bits]"; use_modulo "Use Modulo"; modulo "Count Modulo"; SpecifyClock "Specify Clock"; direction "Counter Direction"; use_sload "Use Synchronous Load Ports (data, sload)"; use_sset "Use Synchronous Set Port (sset)"; svalue "Set Value"; use_clk_ena "Use Clock Enable Port (clk_ena)"; use_ena "Use Counter Enable Port (ena)"; use_sclr "Use Synchronous Clear Port (sclr)"; pipeline_display "Number Of Pipeline Stages (Calculated)"
      mask help: For each cycle, the counter increments or decrements its output by the smallest amount that can be represented by the selected bus type.
      mask init:
      | alt_dspbuilder_init('BlockFactory', 'com.altera.dspbuilder.blockset.arithmetic.Counter', { get_param(gcb, 'BusType') bwl bwr get_param(gcb, 'use_modulo') modulo get_param(gcb, 'SpecifyClock') clock get_param(gcb, 'direction') get_param(gcb, 'use_sload') get_param(gcb, 'use_sset') svalue get_param(gcb, 'use_clk_ena') get_param(gcb, 'use_ena') get_param(gcb, 'use_sclr') pipeline_display });
      settings: CopyFcn=alt_dspbuilder_add_block(gcb, 'BlockFactory', 'com.altera.dspbuilder.blockset.arithmetic.Counter');  DeleteFcn=com.altera.dspbuilder.simulation.Mask.delete(gcb);  UndoDeleteFcn=alt_dspbuilder_add_block(gcb, 'BlockFactory', 'com.altera.dspbuilder.blockset.arithmetic.Counter');  PostSaveFcn=alt_dspbuilder_block_saved(gcb);  NameChangeFcn=alt_dspbuilder_block_renamed(gcb);
      mask Help: helpview(char(com.altera.dspbuilder.simulation.Cache.getBlockTemplate('BlockFactory', 'com.altera.dspbuilder.blockset.arithmetic.Counter').getHelpFile))
      mask StyleString: popup(Signed Integer|Unsigned Integer|Signed Fractional|Unsigned Fractional),edit,edit,checkbox,edit,checkbox,edit,popup(Increment|Decrement|Use Direction Port (updown)),checkbox,checkbox,edit,checkbox,checkbox,checkbox,edit
      mask CallbackString: alt_dspbuilder_update_gui('BlockFactory', 'com.altera.dspbuilder.blockset.arithmetic.Counter', 'BusType', 0);|||alt_dspbuilder_update_gui('BlockFactory', 'com.altera.dspbuilder.blockset.arithmetic.Counter', 'use_modulo', 3);||alt_dspbuilder_update_gui('BlockFactory', 'com.altera.dspbuilder.blockset.arithmetic.Counter', 'SpecifyClock', 5);||alt_dspbuilder_update_gui('BlockFactory', 'com.altera.dspbuilder.blockset.arithmetic.Counter', 'direction', 7);|alt_dspbuilder_update_gui('BlockFactory', 'com.altera.dspbuilder.blockset.arithmetic.Counter', 'use_sload', 8);|alt_dspbuilder_update_gui('BlockFactory', 'com.altera.dspbuilder.blockset.arithmetic.Counter', 'use_sset', 9);||alt_dspbuilder_update_gui('BlockFactory', 'com.altera.dspbuilder.blockset.arithmetic.Counter', 'use_clk_ena', 11);|alt_dspbuilder_update_gui('BlockFactory', 'com.altera.dspbuilder.blockset.arithmetic.Counter', 'use_ena', 12);|alt_dspbuilder_update_gui('BlockFactory', 'com.altera.dspbuilder.blockset.arithmetic.Counter', 'use_sclr', 13);|
      mask TabNameString: Main,Main,Main,Main,Main,Main,Main,Optional Ports and Settings,Optional Ports and Settings,Optional Ports and Settings,Optional Ports and Settings,Optional Ports and Settings,Optional Ports and Settings,Optional Ports and Settings,Optional Ports and Settings
      mask Display:
      | port_label('output', 1, 'q(7:0)');
      | disp('mod255')
  DSP Block : S-Function  LoadFcn=alt_dspbuilder_load_block(gcb, 'BlockFactory', 'com.altera.dspbuilder.blockset.arithmetic.MultiplyAddStratixIII');  FunctionName=sGeneric  Parameters=multipliers BusType bwlA bwrA inputWidthACalc bwlB bwrB inputWidthBCalc shift_mode use_shiftout mult1_direction mult3_direction accumulator accum_direction use_accum_sload okForChainoutCalc chainout_adder use_chainout use_zero_chainout full_resolution bwlOutfix bwrOutfix bwrMultCalc bwlMultCalc bwrOutCalc bwlOutCalc outputWidthCalc output_msb single_dsp_block support_rounding_saturation output_lsb width_msb output_rounding_possible output_round_type output_rounding width_saturate_sign output_saturation_possible output_saturate_type output_saturation use_overflow port_output_is_overflow register_data_inputs register_multiplier register_adder reg_chainout reg_shiftout model_is_delayed use_ena use_aclr or_aclr_inputs pipeline_display  EnableBusSupport=off  mask(Stratix III DSP Block AlteraBlockset){multipliers=2, BusType=Signed Integer, bwlA=8, bwrA=0, inputWidthACalc=8, bwlB=8, bwrB=0, inputWidthBCalc=8, shift_mode=off, use_shiftout=off, mult1_direction=ADD, mult3_direction=ADD, accumulator=off, accum_direction=ADD, use_accum_sload=off, okForChainoutCalc=0, chainout_adder=off, use_chainout=off, use_zero_chainout=off, full_resolution=on, bwlOutfix=8, bwrOutfix=0, bwrMultCalc=0, bwlMultCalc=17, bwrOutCalc=0, bwlOutCalc=17, outputWidthCalc=17, output_msb=17, single_dsp_block=1, support_rounding_saturation=0, output_lsb=0, width_msb=17, output_rounding_possible=0, output_round_type=None (truncate), output_rounding=0, width_saturate_sign=0, output_saturation_possible=0, output_saturate_type=None (wrap), output_saturation=0, use_overflow=off, port_output_is_overflow=0, register_data_inputs=on, register_multiplier=on, register_adder=on, reg_chainout=on, reg_shiftout=on, model_is_delayed=1, use_ena=off, use_aclr=off, or_aclr_inputs=on, pipeline_display=3}
      mask prompts: multipliers "Number of Multipliers (1-4)"; BusType "Bus Type"; bwlA "a Inputs [Number Of Bits].[]"; bwrA "a Inputs [].[Number Of Bits]"; inputWidthACalc "Calculated Input A bitwidth"; bwlB "b Inputs [Number Of Bits].[]"; bwrB "b Inputs [].[Number Of Bits]"; inputWidthBCalc "Calculated Input B bitwidth"; shift_mode "Connect Multiplier Input a to shiftin"; use_shiftout "Use Shiftout from a Input of Last Multiplier (shiftouta)"; mult1_direction "Output Operation on First Multiplier Pair"; mult3_direction "Output Operation on Second Multiplier Pair"; accumulator "Enable Accumulator Mode"; accum_direction "Accumulator Direction"; use_accum_sload "Use Accumulator Synchronous Load Input (accum_sload)"; okForChainoutCalc "Calculated condition for use of chainout"; chainout_adder "Use Chainout Adder Input (chainin)"; use_chainout "Use Chainout Adder Output (chainout)"; use_zero_chainout "Use Zero Chainout Input (zero_chainout)"; full_resolution "Full Resolution for Output Result"; bwlOutfix "Output [Number Of Bits].[]"; bwrOutfix "Output [].[Number Of Bits]"; bwrMultCalc "Calculated Multipliers [].[Number Of Bits]"; bwlMultCalc "Calculated Multipliers [Number Of Bits].[]"; bwrOutCalc "Calculated Output [].[Number Of Bits]"; bwlOutCalc "Calculated Output [Number Of Bits].[]"; outputWidthCalc "Calculated Output bitwidth"; output_msb "MSB of output, ignoring truncation/rounding"; single_dsp_block "Whether operation fits into a single 18x18 DSP block"; support_rounding_saturation "Whether to support rounding and saturation at all"; output_lsb "Number of fractional bits to remove"; width_msb "Number of bits from the MSB (before saturation) to the LSB (after rounding)"; output_rounding_possible "Whether could use first rounding block"; output_round_type "Output Rounding Operation Type"; output_rounding "Whether to use first rounding block"; width_saturate_sign "Saturate position"; output_saturation_possible "Whether output saturation would make sense"; output_saturate_type "Output Saturation Operation Type"; output_saturation "Whether to use first saturation block"; use_overflow "Use Output Overflow Port (overflow)"; port_output_is_overflow "Whether to provide output pin overflow"; register_data_inputs "Register Data Inputs to the Multiplier(s) (always on if shiftin mode)"; register_multiplier "Register Output of the Multiplier"; register_adder "Register Output of the Adder (always on if accumulating)"; reg_chainout "Register Chainout Adder (if used)"; reg_shiftout "Register Shiftout (if used)"; model_is_delayed "Whether model is direct-feedthrough or delayed"; use_ena "Use Enable Port (ena) (if using registers)"; use_aclr "Use Asynchronous Clear Port (aclr) (if using registers)"; or_aclr_inputs "'OR' Asynchronous Clear Input with Global Aclr"; pipeline_display "Number Of Pipeline Stages (Calculated)"
      mask help:
      | The DSP block consists of one to four multipliers feeding a parallel adder. It is equivalent to the Multiply Add block but exposes extra features (including chaining) that are currently available only on Stratix III, Stratix IV and Arria II GX DSP blocks.
      |
      | The DSP block accepts one to four pairs of multiplier inputs a and b. The operands in each pair are multiplied together. The second and fourth multiplier outputs can optionally be added or subtracted from the total.
      |
      | If there are four multipliers and the input bit widths are both less than or equal to 18, you can optionally enable a chainout adder output (chainout) instead of the normal output (res).
      |
      | If there are four multipliers and the input bit widths are both equal to 18, you can enable a chainout adder input (chainin). This chainin port can only be driven from the chainout output of a DSP block at the preceding stage.
      |
      | See the DSP Builder Help or the Quartus II altmult_add Megafunction for full documentation.
      mask init:
      | alt_dspbuilder_init('BlockFactory', 'com.altera.dspbuilder.blockset.arithmetic.MultiplyAddStratixIII', { get_param(gcb, 'multipliers') get_param(gcb, 'BusType') bwlA bwrA inputWidthACalc bwlB bwrB inputWidthBCalc get_param(gcb, 'shift_mode') get_param(gcb, 'use_shiftout') get_param(gcb, 'mult1_direction') get_param(gcb, 'mult3_direction') get_param(gcb, 'accumulator') accum_direction get_param(gcb, 'use_accum_sload') okForChainoutCalc get_param(gcb, 'chainout_adder') get_param(gcb, 'use_chainout') get_param(gcb, 'use_zero_chainout') get_param(gcb, 'full_resolution') bwlOutfix bwrOutfix get_param(gcb, 'bwrMultCalc') get_param(gcb, 'bwlMultCalc') bwrOutCalc bwlOutCalc outputWidthCalc get_param(gcb, 'output_msb') get_param(gcb, 'single_dsp_block') get_param(gcb, 'support_rounding_saturation') output_lsb width_msb get_param(gcb, 'output_rounding_possible') output_round_type get_param(gcb, 'output_rounding') width_saturate_sign get_param(gcb, 'output_saturation_possible') get_param(gcb, 'output_saturate_type') get_param(gcb, 'output_saturation') get_param(gcb, 'use_overflow') get_param(gcb, 'port_output_is_overflow') get_param(gcb, 'register_data_inputs') get_param(gcb, 'register_multiplier') get_param(gcb, 'register_adder') get_param(gcb, 'reg_chainout') get_param(gcb, 'reg_shiftout') model_is_delayed get_param(gcb, 'use_ena') get_param(gcb, 'use_aclr') get_param(gcb, 'or_aclr_inputs') pipeline_display });
      settings: CopyFcn=alt_dspbuilder_add_block(gcb, 'BlockFactory', 'com.altera.dspbuilder.blockset.arithmetic.MultiplyAddStratixIII');  DeleteFcn=com.altera.dspbuilder.simulation.Mask.delete(gcb);  UndoDeleteFcn=alt_dspbuilder_add_block(gcb, 'BlockFactory', 'com.altera.dspbuilder.blockset.arithmetic.MultiplyAddStratixIII');  PostSaveFcn=alt_dspbuilder_block_saved(gcb);  NameChangeFcn=alt_dspbuilder_block_renamed(gcb);
      mask Help: helpview(char(com.altera.dspbuilder.simulation.Cache.getBlockTemplate('BlockFactory', 'com.altera.dspbuilder.blockset.arithmetic.MultiplyAddStratixIII').getHelpFile))
      mask StyleString: popup(1|2|3|4),popup(Signed Integer|Unsigned Integer|Signed Fractional|Unsigned Fractional),edit,edit,edit,edit,edit,edit,checkbox,checkbox,popup(ADD|SUB),popup(ADD|SUB),checkbox,popup(ADD|SUB),checkbox,edit,checkbox,checkbox,checkbox,checkbox,edit,edit,edit,edit,edit,edit,edit,edit,edit,edit,edit,edit,edit,popup(None (truncate)|Nearest Integer|Nearest Even),edit,edit,edit,popup(None (wrap)|Symmetric|Asymmetric),edit,checkbox,edit,checkbox,checkbox,checkbox,checkbox,checkbox,edit,checkbox,checkbox,checkbox,edit
      mask CallbackString: alt_dspbuilder_update_gui('BlockFactory', 'com.altera.dspbuilder.blockset.arithmetic.MultiplyAddStratixIII', 'multipliers', 0);|alt_dspbuilder_update_gui('BlockFactory', 'com.altera.dspbuilder.blockset.arithmetic.MultiplyAddStratixIII', 'BusType', 1);|||||||alt_dspbuilder_update_gui('BlockFactory', 'com.altera.dspbuilder.blockset.arithmetic.MultiplyAddStratixIII', 'shift_mode', 8);|alt_dspbuilder_update_gui('BlockFactory', 'com.altera.dspbuilder.blockset.arithmetic.MultiplyAddStratixIII', 'use_shiftout', 9);|alt_dspbuilder_update_gui('BlockFactory', 'com.altera.dspbuilder.blockset.arithmetic.MultiplyAddStratixIII', 'mult1_direction', 10);|alt_dspbuilder_update_gui('BlockFactory', 'com.altera.dspbuilder.blockset.arithmetic.MultiplyAddStratixIII', 'mult3_direction', 11);|alt_dspbuilder_update_gui('BlockFactory', 'com.altera.dspbuilder.blockset.arithmetic.MultiplyAddStratixIII', 'accumulator', 12);||alt_dspbuilder_update_gui('BlockFactory', 'com.altera.dspbuilder.blockset.arithmetic.MultiplyAddStratixIII', 'use_accum_sload', 14);||alt_dspbuilder_update_gui('BlockFactory', 'com.altera.dspbuilder.blockset.arithmetic.MultiplyAddStratixIII', 'chainout_adder', 16);|alt_dspbuilder_update_gui('BlockFactory', 'com.altera.dspbuilder.blockset.arithmetic.MultiplyAddStratixIII', 'use_chainout', 17);|alt_dspbuilder_update_gui('BlockFactory', 'com.altera.dspbuilder.blockset.arithmetic.MultiplyAddStratixIII', 'use_zero_chainout', 18);|alt_dspbuilder_update_gui('BlockFactory', 'com.altera.dspbuilder.blockset.arithmetic.MultiplyAddStratixIII', 'full_resolution', 19);|||alt_dspbuilder_update_gui('BlockFactory', 'com.altera.dspbuilder.blockset.arithmetic.MultiplyAddStratixIII', 'bwrMultCalc', 22);|alt_dspbuilder_update_gui('BlockFactory', 'com.altera.dspbuilder.blockset.arithmetic.MultiplyAddStratixIII', 'bwlMultCalc', 23);||||alt_dspbuilder_update_gui('BlockFactory', 'com.altera.dspbuilder.blockset.arithmetic.MultiplyAddStratixIII', 'output_msb', 27);|alt_dspbuilder_update_gui('BlockFactory', 'com.altera.dspbuilder.blockset.arithmetic.MultiplyAddStratixIII', 'single_dsp_block', 28);|alt_dspbuilder_update_gui('BlockFactory', 'com.altera.dspbuilder.blockset.arithmetic.MultiplyAddStratixIII', 'support_rounding_saturation', 29);|||alt_dspbuilder_update_gui('BlockFactory', 'com.altera.dspbuilder.blockset.arithmetic.MultiplyAddStratixIII', 'output_rounding_possible', 32);||alt_dspbuilder_update_gui('BlockFactory', 'com.altera.dspbuilder.blockset.arithmetic.MultiplyAddStratixIII', 'output_rounding', 34);||alt_dspbuilder_update_gui('BlockFactory', 'com.altera.dspbuilder.blockset.arithmetic.MultiplyAddStratixIII', 'output_saturation_possible', 36);|alt_dspbuilder_update_gui('BlockFactory', 'com.altera.dspbuilder.blockset.arithmetic.MultiplyAddStratixIII', 'output_saturate_type', 37);|alt_dspbuilder_update_gui('BlockFactory', 'com.altera.dspbuilder.blockset.arithmetic.MultiplyAddStratixIII', 'output_saturation', 38);|alt_dspbuilder_update_gui('BlockFactory', 'com.altera.dspbuilder.blockset.arithmetic.MultiplyAddStratixIII', 'use_overflow', 39);|alt_dspbuilder_update_gui('BlockFactory', 'com.altera.dspbuilder.blockset.arithmetic.MultiplyAddStratixIII', 'port_output_is_overflow', 40);|alt_dspbuilder_update_gui('BlockFactory', 'com.altera.dspbuilder.blockset.arithmetic.MultiplyAddStratixIII', 'register_data_inputs', 41);|alt_dspbuilder_update_gui('BlockFactory', 'com.altera.dspbuilder.blockset.arithmetic.MultiplyAddStratixIII', 'register_multiplier', 42);|alt_dspbuilder_update_gui('BlockFactory', 'com.altera.dspbuilder.blockset.arithmetic.MultiplyAddStratixIII', 'register_adder', 43);|alt_dspbuilder_update_gui('BlockFactory', 'com.altera.dspbuilder.blockset.arithmetic.MultiplyAddStratixIII', 'reg_chainout', 44);|alt_dspbuilder_update_gui('BlockFactory', 'com.altera.dspbuilder.blockset.arithmetic.MultiplyAddStratixIII', 'reg_shiftout', 45);||alt_dspbuilder_update_gui('BlockFactory', 'com.altera.dspbuilder.blockset.arithmetic.MultiplyAddStratixIII', 'use_ena', 47);|alt_dspbuilder_update_gui('BlockFactory', 'com.altera.dspbuilder.blockset.arithmetic.MultiplyAddStratixIII', 'use_aclr', 48);|alt_dspbuilder_update_gui('BlockFactory', 'com.altera.dspbuilder.blockset.arithmetic.MultiplyAddStratixIII', 'or_aclr_inputs', 49);|
      mask TabNameString: Inputs,Inputs,Inputs,Inputs,Inputs,Inputs,Inputs,Inputs,Inputs,Inputs,Behavior,Behavior,Behavior,Behavior,Behavior,Behavior,Behavior,Behavior,Behavior,Optional Bus Sizing,Optional Bus Sizing,Optional Bus Sizing,Optional Bus Sizing,Optional Bus Sizing,Optional Bus Sizing,Optional Bus Sizing,Optional Bus Sizing,Optional Bus Sizing,Optional Bus Sizing,Optional Bus Sizing,Optional Bus Sizing,Optional Bus Sizing,Optional Bus Sizing,Optional Bus Sizing,Optional Bus Sizing,Optional Bus Sizing,Optional Bus Sizing,Optional Bus Sizing,Optional Bus Sizing,Optional Bus Sizing,Optional Bus Sizing,Pipeline and Control,Pipeline and Control,Pipeline and Control,Pipeline and Control,Pipeline and Control,Pipeline and Control,Pipeline and Control,Pipeline and Control,Pipeline and Control,Pipeline and Control
      mask Display:
      | port_label('input', 1, 'a0(7:0)');
      | port_label('input', 2, 'b0(7:0)');
      | port_label('input', 3, 'a1(7:0)');
      | port_label('input', 4, 'b1(7:0)');
      | port_label('output', 1, 'res(16:0)');
      | 
      | disp('res = a0 X b0 + a1 X b1');
  Decoder : S-Function  LoadFcn=alt_dspbuilder_load_block(gcb, 'BlockFactory', 'com.altera.dspbuilder.blockset.gatecontrol.Decoder');  FunctionName=sGeneric  Parameters=BusType bwl bwr registered pipeline_display value  EnableBusSupport=off  mask(Decoder AlteraBlockset){BusType=Unsigned Integer, bwl=2, bwr=2, registered=on, pipeline_display=1, value=1}
      mask prompts: BusType "Input Bus Type"; bwl "[Number Of Bits].[]"; bwr "[].[Number Of Bits]"; registered "Register Output"; pipeline_display "Number Of Pipeline Stages (Calculated)"; value "Decoded Value"
      mask help:
      | Compares the input value against the specified decoded value. If the values match, the block outputs a 1, if they do not match it outputs a 0.
      | If the specified value is not representable in the data type of the input bus, it is truncated to the data type of the input bus. For example: 5 (binary 101) as a 2 bit unsigned integer would result in 1 (binary 01)
      mask init:
      | alt_dspbuilder_init('BlockFactory', 'com.altera.dspbuilder.blockset.gatecontrol.Decoder', { get_param(gcb, 'BusType') bwl bwr registered pipeline_display value });
      settings: CopyFcn=alt_dspbuilder_add_block(gcb, 'BlockFactory', 'com.altera.dspbuilder.blockset.gatecontrol.Decoder');  DeleteFcn=com.altera.dspbuilder.simulation.Mask.delete(gcb);  UndoDeleteFcn=alt_dspbuilder_add_block(gcb, 'BlockFactory', 'com.altera.dspbuilder.blockset.gatecontrol.Decoder');  PostSaveFcn=alt_dspbuilder_block_saved(gcb);  NameChangeFcn=alt_dspbuilder_block_renamed(gcb);
      mask Help: helpview(char(com.altera.dspbuilder.simulation.Cache.getBlockTemplate('BlockFactory', 'com.altera.dspbuilder.blockset.gatecontrol.Decoder').getHelpFile))
      mask StyleString: popup(Signed Integer|Unsigned Integer|Signed Fractional|Unsigned Fractional),edit,edit,checkbox,edit,edit
      mask CallbackString: alt_dspbuilder_update_gui('BlockFactory', 'com.altera.dspbuilder.blockset.gatecontrol.Decoder', 'BusType', 0);|||||
      mask Display:
      | port_label('input', 1, 'in(1:0)');
      | port_label('output', 1, 'match');
  Delay : S-Function  LoadFcn=alt_dspbuilder_load_block(gcb, 'BlockFactory', 'com.altera.dspbuilder.blockset.storage.Delay');  FunctionName=sGeneric  Parameters=pipeline pipeline_display ClockPhase use_ena use_sclr allowFloatingPointOverride logOutputs logFile use_init reset_value  EnableBusSupport=off  mask(Delay AlteraBlockset){pipeline=1, pipeline_display=1, ClockPhase=1, use_ena=off, use_sclr=off, allowFloatingPointOverride=on, logOutputs=off, logFile=D:\\allblocks%5Falteradspbuilder2_Delay.fixedpointlog, use_init=off, reset_value=1}
      mask prompts: pipeline "Number Of Pipeline Stages"; pipeline_display "Number Of Pipeline Stages (Calculated)"; ClockPhase "Clock Phase Selection"; use_ena "Use Enable Port (ena)"; use_sclr "Use Synchronous Clear port (sclr)"; allowFloatingPointOverride "Allow Floating Point Override For This Block"; use_init "Reset To Constant (Non-Zero) Value"; reset_value "Reset Value"
      mask help: Delays the incoming data by an amount specified by the number of pipeline stages. The Delay block accepts any data type as inputs.
      mask init:
      | alt_dspbuilder_init('BlockFactory', 'com.altera.dspbuilder.blockset.storage.Delay', { pipeline pipeline_display ClockPhase use_ena use_sclr allowFloatingPointOverride logOutputs logFile get_param(gcb, 'use_init') reset_value });
      settings: CopyFcn=alt_dspbuilder_add_block(gcb, 'BlockFactory', 'com.altera.dspbuilder.blockset.storage.Delay');  DeleteFcn=com.altera.dspbuilder.simulation.Mask.delete(gcb);  UndoDeleteFcn=alt_dspbuilder_add_block(gcb, 'BlockFactory', 'com.altera.dspbuilder.blockset.storage.Delay');  PostSaveFcn=alt_dspbuilder_block_saved(gcb);  NameChangeFcn=alt_dspbuilder_block_renamed(gcb);
      mask Help: helpview(char(com.altera.dspbuilder.simulation.Cache.getBlockTemplate('BlockFactory', 'com.altera.dspbuilder.blockset.storage.Delay').getHelpFile))
      mask CallbackString: ||||||||alt_dspbuilder_update_gui('BlockFactory', 'com.altera.dspbuilder.blockset.storage.Delay', 'use_init', 8);|
      mask TabNameString: Main,Main,Optional Ports,Optional Ports,Optional Ports,Optional Ports,Optional Ports,Optional Ports,Initialization,Initialization
      mask Display: disp('z^{-1}','texmode','on');
  Demultiplexer : S-Function  LoadFcn=alt_dspbuilder_load_block(gcb, 'BlockFactory', 'com.altera.dspbuilder.blockset.gatecontrol.Demultiplexer');  FunctionName=sGeneric  Parameters=numOutputs pipeline_display use_ena use_sclr allowFloatingPointOverride logOutputs logFile  EnableBusSupport=off  mask(Demultiplexer AlteraBlockset){numOutputs=6, pipeline_display=1, use_ena=off, use_sclr=off, allowFloatingPointOverride=on, logOutputs=off, logFile=D:\\allblocks%5Falteradspbuilder2_Demultiplexer%3A%3Aq.fixedpointlog,D:\\allblocks%5Falteradspbuilder2_Demultiplexer%3A%3Aq.fixedpointlog,D:\\allblocks%5Falteradspbuilder2_Demultiplexer%3A%3Aq.fixedpointlog,D:\\allblocks%5Falteradspbuilder2_Demultiplexer%3A%3Aq.fixedpointlog,D:\\allblocks%5Falteradspbuilder2_Demultiplexer%3A%3Aq.fixedpointlog,D:\\allblocks%5Falteradspbuilder2_Demultiplexer%3A%3Aq.fixedpointlog,}
      mask prompts: numOutputs "Number of Output Data Lines"; pipeline_display "Number Of Pipeline Stages (Calculated)"; use_ena "Use Enable Port (ena)"; use_sclr "Use Synchronous Clear Port (sclr)"; allowFloatingPointOverride "Allow Floating Point Override For This Block"
      mask help:
      | A one-to-N demultiplexer that outputs the value of the input (d) to the selected output. All other outputs will remain constant.
      | The select input (sel) is of type Unsigned Integer.
      mask init:
      | alt_dspbuilder_init('BlockFactory', 'com.altera.dspbuilder.blockset.gatecontrol.Demultiplexer', { numOutputs pipeline_display use_ena use_sclr allowFloatingPointOverride logOutputs logFile });
      settings: CopyFcn=alt_dspbuilder_add_block(gcb, 'BlockFactory', 'com.altera.dspbuilder.blockset.gatecontrol.Demultiplexer');  DeleteFcn=com.altera.dspbuilder.simulation.Mask.delete(gcb);  UndoDeleteFcn=alt_dspbuilder_add_block(gcb, 'BlockFactory', 'com.altera.dspbuilder.blockset.gatecontrol.Demultiplexer');  PostSaveFcn=alt_dspbuilder_block_saved(gcb);  NameChangeFcn=alt_dspbuilder_block_renamed(gcb);
      mask Help: helpview(char(com.altera.dspbuilder.simulation.Cache.getBlockTemplate('BlockFactory', 'com.altera.dspbuilder.blockset.gatecontrol.Demultiplexer').getHelpFile))
      mask TabNameString: Main,Main,Optional Ports,Optional Ports,Optional Ports,Optional Ports,Optional Ports
      mask Display:
      | port_label('input', 1, 'd');
      | port_label('input', 2, 'sel(2:0)');
      | port_label('output', 1, '0');
      | port_label('output', 2, '1');
      | port_label('output', 3, '2');
      | port_label('output', 4, '3');
      | port_label('output', 5, '4');
      | port_label('output', 6, '5');
      | plot([1 0.25 0 0 0.25 1 1], [0 0 0.2 0.8 1 1 0])
      | disp('DEMUX');
  Differentiator : S-Function  LoadFcn=alt_dspbuilder_load_block(gcb, 'BlockFactory', 'com.altera.dspbuilder.blockset.arithmetic.Differentiator');  FunctionName=sGeneric  Parameters=bwl depth pipeline_display use_ena use_sclr allowFloatingPointOverride logOutputs logFile  EnableBusSupport=off  mask(Differentiator AlteraBlockset){bwl=20, depth=1, pipeline_display=1, use_ena=on, use_sclr=on, allowFloatingPointOverride=on, logOutputs=off, logFile=D:\\allblocks%5Falteradspbuilder2_Differentiator.fixedpointlog}
      mask prompts: bwl "Number Of Bits"; pipeline_display "Number Of Pipeline Stages (Calculated)"; use_ena "Use Enable Port (ena)"; use_sclr "Use Synchronous Clear Port (sclr)"; allowFloatingPointOverride "Allow Floating Point Override For This Block"
      mask help:
      | Signed integer differentiator with the equation:
      |   q(n) = d(n) - d(n-D) where D is the delay parameter.
      mask init:
      | alt_dspbuilder_init('BlockFactory', 'com.altera.dspbuilder.blockset.arithmetic.Differentiator', { bwl depth pipeline_display get_param(gcb, 'use_ena') get_param(gcb, 'use_sclr') allowFloatingPointOverride logOutputs logFile });
      settings: CopyFcn=alt_dspbuilder_add_block(gcb, 'BlockFactory', 'com.altera.dspbuilder.blockset.arithmetic.Differentiator');  DeleteFcn=com.altera.dspbuilder.simulation.Mask.delete(gcb);  UndoDeleteFcn=alt_dspbuilder_add_block(gcb, 'BlockFactory', 'com.altera.dspbuilder.blockset.arithmetic.Differentiator');  PostSaveFcn=alt_dspbuilder_block_saved(gcb);  NameChangeFcn=alt_dspbuilder_block_renamed(gcb);
      mask Help: helpview(char(com.altera.dspbuilder.simulation.Cache.getBlockTemplate('BlockFactory', 'com.altera.dspbuilder.blockset.arithmetic.Differentiator').getHelpFile))
      mask CallbackString: |||alt_dspbuilder_update_gui('BlockFactory', 'com.altera.dspbuilder.blockset.arithmetic.Differentiator', 'use_ena', 3);|alt_dspbuilder_update_gui('BlockFactory', 'com.altera.dspbuilder.blockset.arithmetic.Differentiator', 'use_sclr', 4);|||
      mask TabNameString: Main,Main,Main,Optional Ports,Optional Ports,Optional Ports,Optional Ports,Optional Ports
      mask Display:
      | port_label('input', 1, 'd(19:0)');
      | port_label('input', 2, 'ena');
      | port_label('input', 3, 'sclr');
      | port_label('output', 1, 'q(19:0)');
      | disp('1 - z^{-1}', 'texmode', 'on');
  Display Pipeline Depth : S-Function  LoadFcn=alt_dspbuilder_load_block(gcb, 'BlockFactory', 'com.altera.dspbuilder.blockset.altlab.DisplayLatency');  FunctionName=sNoOp  Parameters=DisplayLatencyOnBlocks  EnableBusSupport=off  mask(Display Latency AlteraBlockset){DisplayLatencyOnBlocks=off}
      mask prompts: DisplayLatencyOnBlocks "Display Pipeline Depth"
      mask help:
      | Tcontrols whether the pipeline depth is displayed on primitive blocks.
      | You can change the display mode by double-clicking on the block. When set, the current pipeline depth is displayed at the top right corner of each block that adds latency to your design. The currently selected mode is shown on the Display Pipeline Depth block symbol.
      | Changing modes causes a Simulink display update which may be slow for very large designs.
      mask init:
      | alt_dspbuilder_init('BlockFactory', 'com.altera.dspbuilder.blockset.altlab.DisplayLatency', { DisplayLatencyOnBlocks });
      settings: CopyFcn=alt_dspbuilder_add_block(gcb, 'BlockFactory', 'com.altera.dspbuilder.blockset.altlab.DisplayLatency');  DeleteFcn=com.altera.dspbuilder.simulation.Mask.delete(gcb);  UndoDeleteFcn=alt_dspbuilder_add_block(gcb, 'BlockFactory', 'com.altera.dspbuilder.blockset.altlab.DisplayLatency');  PostSaveFcn=alt_dspbuilder_block_saved(gcb);  NameChangeFcn=alt_dspbuilder_block_renamed(gcb);
      settings: OpenFcn=|
      | com.altera.dspbuilder.simulation.Mask.simpleInit('BlockFactory', 'com.altera.dspbuilder.blockset.altlab.DisplayLatency', bdroot(gcb), gcb);
      | alt_dspbuilder_display_latency_switch(gcb)
      mask Help: helpview(char(com.altera.dspbuilder.simulation.Cache.getBlockTemplate('BlockFactory', 'com.altera.dspbuilder.blockset.altlab.DisplayLatency').getHelpFile))
      mask Display: fprintf('Pipeline Depth Display Off');
  Divider : S-Function  LoadFcn=alt_dspbuilder_load_block(gcb, 'BlockFactory', 'com.altera.dspbuilder.blockset.arithmetic.Divider');  FunctionName=sGeneric  Parameters=BusType bwl bwr pipeline pipeline_display use_ena use_aclr  EnableBusSupport=off  mask(Divider AlteraBlockset){BusType=Signed Integer, bwl=8, bwr=0, pipeline=0, pipeline_display=0, use_ena=off, use_aclr=off}
      mask prompts: BusType "Bus Type"; bwl "Input [Number Of Bits].[]"; bwr "Input [].[Number Of Bits]"; pipeline "Number of Pipeline Stages"; pipeline_display "Number Of Pipeline Stages (Calculated)"; use_ena "Use Enable Port (ena)"; use_aclr "Use Aynchronous Clear Port (aclr)"
      mask help:
      | Takes a numerator and a denominator and returns the quotient and a remainder using the equation:
      |    a = b * q + r
      | q and r are undefined if b is zero.
      |
      | Dividing a maximally negative number by a minimally negative one (-1 if using signed integers), outputs a truncated answer.
      | The numerator and denominator inputs can have different widths but are converted to the specified bit width.
      mask init:
      | alt_dspbuilder_init('BlockFactory', 'com.altera.dspbuilder.blockset.arithmetic.Divider', { get_param(gcb, 'BusType') bwl bwr pipeline pipeline_display use_ena use_aclr });
      settings: CopyFcn=alt_dspbuilder_add_block(gcb, 'BlockFactory', 'com.altera.dspbuilder.blockset.arithmetic.Divider');  DeleteFcn=com.altera.dspbuilder.simulation.Mask.delete(gcb);  UndoDeleteFcn=alt_dspbuilder_add_block(gcb, 'BlockFactory', 'com.altera.dspbuilder.blockset.arithmetic.Divider');  PostSaveFcn=alt_dspbuilder_block_saved(gcb);  NameChangeFcn=alt_dspbuilder_block_renamed(gcb);
      mask Help: helpview(char(com.altera.dspbuilder.simulation.Cache.getBlockTemplate('BlockFactory', 'com.altera.dspbuilder.blockset.arithmetic.Divider').getHelpFile))
      mask StyleString: popup(Signed Integer|Unsigned Integer|Signed Fractional|Unsigned Fractional),edit,edit,edit,edit,checkbox,checkbox
      mask CallbackString: alt_dspbuilder_update_gui('BlockFactory', 'com.altera.dspbuilder.blockset.arithmetic.Divider', 'BusType', 0);||||||
      mask TabNameString: Main,Main,Main,Main,Main,Optional Ports,Optional Ports
      mask Display:
      | port_label('input', 1, 'a(7:0)');
      | port_label('input', 2, 'b(7:0)');
      | port_label('output', 1, 'q(7:0)');
      | port_label('output', 2, 'r(7:0)');
      | disp('a = b X q + r');
  Down Sampling : S-Function  LoadFcn=alt_dspbuilder_load_block(gcb, 'BlockFactory', 'com.altera.dspbuilder.blockset.storage.DownSampling');  FunctionName=sGeneric  Parameters=rate allowFloatingPointOverride logOutputs logFile  EnableBusSupport=off  mask(Down Sampling AlteraBlockset){rate=100, allowFloatingPointOverride=on, logOutputs=off, logFile=D:\\allblocks%5Falteradspbuilder2_Down+Sampling.fixedpointlog}
      mask prompts: rate "Down-Sampling Rate"; allowFloatingPointOverride "Allow Floating Point Override For This Block"
      mask help:
      | Decreases the output sample rate from the input sample rate.
      | The output data is sampled at every Nth cycle where N is the down sampling rate.
      | The output data is then held constant for the next N input cycles.
      mask init:
      | alt_dspbuilder_init('BlockFactory', 'com.altera.dspbuilder.blockset.storage.DownSampling', { rate allowFloatingPointOverride logOutputs logFile });
      settings: CopyFcn=alt_dspbuilder_add_block(gcb, 'BlockFactory', 'com.altera.dspbuilder.blockset.storage.DownSampling');  DeleteFcn=com.altera.dspbuilder.simulation.Mask.delete(gcb);  UndoDeleteFcn=alt_dspbuilder_add_block(gcb, 'BlockFactory', 'com.altera.dspbuilder.blockset.storage.DownSampling');  PostSaveFcn=alt_dspbuilder_block_saved(gcb);  NameChangeFcn=alt_dspbuilder_block_renamed(gcb);
      mask Help: helpview(char(com.altera.dspbuilder.simulation.Cache.getBlockTemplate('BlockFactory', 'com.altera.dspbuilder.blockset.storage.DownSampling').getHelpFile))
      mask Display:
      | port_label('input', 1, 'd');
      | port_label('output', 1, 'q');
      | disp('x{100}','texmode','on');
  Dual-Clock FIFO : S-Function  LoadFcn=alt_dspbuilder_load_block(gcb, 'BlockFactory', 'com.altera.dspbuilder.blockset.storage.DualClockFIFO');  FunctionName=sMultiRate  Parameters=numwords BusType bwl bwr ram_type UseBaseWriteClock UseBaseReadClock use_rdempty use_rdfull use_rdusedw use_wrempty use_wrfull use_wrusedw use_user_aclr register_output use_les_only showahead_mode synchronized allowFloatingPointOverride logOutputs logFile  EnableBusSupport=off  mask(Dual-Clock FIFO AlteraBlockset){numwords=64, BusType=Signed Integer, bwl=8, bwr=0, ram_type=AUTO, UseBaseWriteClock=on, write_clock=, UseBaseReadClock=on, read_clock=, use_rdempty=off, use_rdfull=off, use_rdusedw=off, use_wrempty=off, use_wrfull=off, use_wrusedw=off, use_user_aclr=off, register_output=off, use_les_only=off, showahead_mode=off, synchronized=off, allowFloatingPointOverride=on, logOutputs=off, logFile=D:\\allblocks%5Falteradspbuilder2_Dual-Clock+FIFO.fixedpointlog}
      mask prompts: numwords "Number Of Words In FIFO"; BusType "Data Type"; bwl "[Number Of Bits].[]"; bwr "[].[Number Of Bits]"; ram_type "Memory Block Type"; UseBaseWriteClock "Use Base Clock for Write Side"; write_clock "Write-Side Clock"; UseBaseReadClock "Use Base Clock for Read Side"; read_clock "Read-Side Clock"; use_rdempty "Use Read-Side Synchronised EMPTY Port (rdempty)"; use_rdfull "Use Read-Side Synchronised FULL Port (rdfull)"; use_rdusedw "Use Read-Side Synchronised USEDW Port (rdusedw)"; use_wrempty "Use Write-Side Synchronised EMPTY Port (wrempty)"; use_wrfull "Use Write-Side Synchronised FULL Port (wrfull)"; use_wrusedw "Use Write-Side Synchronised USEDW Port (wrusedw)"; use_user_aclr "Use Asynchronous Clear Port (aclr)"; register_output "Register Output (faster, but larger)"; use_les_only "Implement FIFO With Logic Cells Only"; showahead_mode "Use Show-Ahead Mode of Read Request"; synchronized "Calculated parameter specifying whether the clocks are in sync. Do no edit"; allowFloatingPointOverride "Allow Floating Point Override For This Block"
      mask help:
      | Implements a parameterized dual-clock FIFO buffer controlled by separate read-side and write-side clocks.
      |
      | Note that the Dual-Clock FIFO block simulation in Simulink is functionally equivalent to hardware, but not cycle-accurate.
      mask init:
      | alt_dspbuilder_init('BlockFactory', 'com.altera.dspbuilder.blockset.storage.DualClockFIFO', { numwords get_param(gcb, 'BusType') bwl bwr ram_type get_param(gcb, 'UseBaseWriteClock') write_clock get_param(gcb, 'UseBaseReadClock') read_clock get_param(gcb, 'use_rdempty') get_param(gcb, 'use_rdfull') get_param(gcb, 'use_rdusedw') get_param(gcb, 'use_wrempty') get_param(gcb, 'use_wrfull') get_param(gcb, 'use_wrusedw') get_param(gcb, 'use_user_aclr') register_output use_les_only showahead_mode synchronized allowFloatingPointOverride logOutputs logFile });
      settings: CopyFcn=alt_dspbuilder_add_block(gcb, 'BlockFactory', 'com.altera.dspbuilder.blockset.storage.DualClockFIFO');  DeleteFcn=com.altera.dspbuilder.simulation.Mask.delete(gcb);  UndoDeleteFcn=alt_dspbuilder_add_block(gcb, 'BlockFactory', 'com.altera.dspbuilder.blockset.storage.DualClockFIFO');  PostSaveFcn=alt_dspbuilder_block_saved(gcb);  NameChangeFcn=alt_dspbuilder_block_renamed(gcb);
      mask Help: helpview(char(com.altera.dspbuilder.simulation.Cache.getBlockTemplate('BlockFactory', 'com.altera.dspbuilder.blockset.storage.DualClockFIFO').getHelpFile))
      mask StyleString: edit,popup(Signed Integer|Unsigned Integer|Signed Fractional|Unsigned Fractional),edit,edit,popup(AUTO|M9K|M10K|M20K|MLAB|M144K),checkbox,edit,checkbox,edit,checkbox,checkbox,checkbox,checkbox,checkbox,checkbox,checkbox,checkbox,checkbox,checkbox,checkbox,checkbox,checkbox,edit
      mask CallbackString: |alt_dspbuilder_update_gui('BlockFactory', 'com.altera.dspbuilder.blockset.storage.DualClockFIFO', 'BusType', 1);||||alt_dspbuilder_update_gui('BlockFactory', 'com.altera.dspbuilder.blockset.storage.DualClockFIFO', 'UseBaseWriteClock', 5);||alt_dspbuilder_update_gui('BlockFactory', 'com.altera.dspbuilder.blockset.storage.DualClockFIFO', 'UseBaseReadClock', 7);||alt_dspbuilder_update_gui('BlockFactory', 'com.altera.dspbuilder.blockset.storage.DualClockFIFO', 'use_rdempty', 9);|alt_dspbuilder_update_gui('BlockFactory', 'com.altera.dspbuilder.blockset.storage.DualClockFIFO', 'use_rdfull', 10);|alt_dspbuilder_update_gui('BlockFactory', 'com.altera.dspbuilder.blockset.storage.DualClockFIFO', 'use_rdusedw', 11);|alt_dspbuilder_update_gui('BlockFactory', 'com.altera.dspbuilder.blockset.storage.DualClockFIFO', 'use_wrempty', 12);|alt_dspbuilder_update_gui('BlockFactory', 'com.altera.dspbuilder.blockset.storage.DualClockFIFO', 'use_wrfull', 13);|alt_dspbuilder_update_gui('BlockFactory', 'com.altera.dspbuilder.blockset.storage.DualClockFIFO', 'use_wrusedw', 14);|alt_dspbuilder_update_gui('BlockFactory', 'com.altera.dspbuilder.blockset.storage.DualClockFIFO', 'use_user_aclr', 15);|||||||
      mask TabNameString: Main,Main,Main,Main,Main,Main,Main,Main,Main,Optional Ports and Settings,Optional Ports and Settings,Optional Ports and Settings,Optional Ports and Settings,Optional Ports and Settings,Optional Ports and Settings,Optional Ports and Settings,Optional Ports and Settings,Optional Ports and Settings,Optional Ports and Settings,Optional Ports and Settings,Optional Ports and Settings,Optional Ports and Settings,Optional Ports and Settings
      mask Display:
      | port_label('input', 1, 'd');
      | port_label('input', 2, 'wrreq');
      | port_label('input', 3, 'rdreq');
      | port_label('output', 1, 'q');
      | disp('DC FIFO');
  Dual-Port RAM : S-Function  LoadFcn=alt_dspbuilder_load_block(gcb, 'BlockFactory', 'com.altera.dspbuilder.blockset.storage.DualRam');  FunctionName=sGeneric  Parameters=numwords BusType bwl bwr memory_type ram_type dont_care initialization init_file init_array register_outputs use_ena ClockPhase allowFloatingPointOverride logOutputs logFile pipeline_display  EnableBusSupport=off  mask(Dual-Port RAM AlteraBlockset){numwords=16, BusType=Signed Integer, bwl=8, bwr=0, memory_type=AUTO, ram_type=DualRAM, dont_care=off, initialization=Blank, init_file=input.hex, init_array=[0:1:15], register_outputs=on, use_ena=off, ClockPhase=1, allowFloatingPointOverride=on, logOutputs=off, logFile=D:\\allblocks%5Falteradspbuilder2_Dual-Port+RAM.fixedpointlog, pipeline_display=2}
      mask prompts: numwords "Number Of Words"; BusType "Data Type"; bwl "[Number Of Bits].[]"; bwr "[].[Number Of Bits]"; memory_type "Memory Block Type"; ram_type "RAM type"; dont_care "Use DONT_CARE when reading from and writing to the same address"; init_file "Input HEX File"; init_array "MATLAB Array"; register_outputs "Register Output Port"; use_ena "Use Enable Port (ena)"; ClockPhase "Clock Phase Selection"; allowFloatingPointOverride "Allow Floating Point Override For This Block"; pipeline_display "Number Of Pipeline Stages (Calculated)"
      mask help:
      | Maps data to an embedded RAM (embedded array block, EAB; or embedded system block, ESB) in Altera devices. The read and write ports are separate.
      |
      | The Simple Dual-Port RAM block accepts any data input type. The input port is always registered and the output port can optionally be registered.
      |
      | The contents of the RAM are pre-initialized to zero by default, but can be specified from an Intel-format Hexadecimal (.hex) file, or from a MATLAB array. You can use the Quartus II software to generate a .hex File which must be in your DSP Builder working directory. If used, the MATLAB array parameter must be a one dimensional MATLAB array with a length less than or equal to the number of words. The array can be specified from the MATLAB workspace or directly in the MATLAB Array entry box.
      |
      | Note that the input address bus must be Unsigned and the clock enable (ena) bypasses any output register. For memory type M-RAM initialization is not possible. For memory type MLAB, output registers will always be used unless 'DONT_CARE' is selected - in which case output registers will be optional.
      |
      | Turning on the DONT_CARE option may give a higher fMAX for your design, especially if the memory is implemented as a MLAB. When this option is on, the output is not double-registered (and therefore, in the case of MLAB implementation, uses fewer external registers), and you gain an extra half-cycle on the output. The default is off, which outputs old data for read-during-write.
      mask init:
      | alt_dspbuilder_init('BlockFactory', 'com.altera.dspbuilder.blockset.storage.DualRam', { numwords get_param(gcb, 'BusType') bwl bwr get_param(gcb, 'memory_type') ram_type dont_care get_param(gcb, 'initialization') init_file init_array register_outputs get_param(gcb, 'use_ena') ClockPhase allowFloatingPointOverride logOutputs logFile pipeline_display });
      settings: CopyFcn=alt_dspbuilder_add_block(gcb, 'BlockFactory', 'com.altera.dspbuilder.blockset.storage.DualRam');  DeleteFcn=com.altera.dspbuilder.simulation.Mask.delete(gcb);  UndoDeleteFcn=alt_dspbuilder_add_block(gcb, 'BlockFactory', 'com.altera.dspbuilder.blockset.storage.DualRam');  PostSaveFcn=alt_dspbuilder_block_saved(gcb);  NameChangeFcn=alt_dspbuilder_block_renamed(gcb);
      mask Help: helpview(char(com.altera.dspbuilder.simulation.Cache.getBlockTemplate('BlockFactory', 'com.altera.dspbuilder.blockset.storage.DualRam').getHelpFile))
      mask StyleString: edit,popup(Inferred|Signed Integer|Unsigned Integer|Signed Fractional|Unsigned Fractional),edit,edit,popup(AUTO|M9K|M10K|M20K|MLAB|M144K),popup(ROM|SingleRAM|DualRAM|TrueDualRAM),checkbox,popup(Blank|From HEX file|From MATLAB array),edit,edit,checkbox,checkbox,edit,checkbox,checkbox,edit,edit
      mask CallbackString: |alt_dspbuilder_update_gui('BlockFactory', 'com.altera.dspbuilder.blockset.storage.DualRam', 'BusType', 1);|||alt_dspbuilder_update_gui('BlockFactory', 'com.altera.dspbuilder.blockset.storage.DualRam', 'memory_type', 4);|||alt_dspbuilder_update_gui('BlockFactory', 'com.altera.dspbuilder.blockset.storage.DualRam', 'initialization', 7);||||alt_dspbuilder_update_gui('BlockFactory', 'com.altera.dspbuilder.blockset.storage.DualRam', 'use_ena', 11);|||||
      mask TabNameString: Main,Main,Main,Main,Main,Main,Main,Initialization,Initialization,Initialization,Registers and Enables,Registers and Enables,Registers and Enables,Registers and Enables,Registers and Enables,Registers and Enables,Registers and Enables
      mask Display:
      | port_label('input', 1, 'd(7:0)');
      | port_label('input', 2, 'rd_add(3:0)');
      | port_label('input', 3, 'wr_add(3:0)');
      | port_label('input', 4, 'wren');
      | port_label('output', 1, 'q_a');
      | fprintf('DPRAM\n(%d x %d)' , 16, 8);
  External RAM : S-Function  StartFcn=alt_dspbuilder_internal_externalRAMWarning  FunctionName=sSinglePortRAM  Parameters=DATA_WIDTH ADDRESS_WIDTH WAIT_STATES_PER_WRITE MAXIMUM_LATENCY SIZE OFFSET  EnableBusSupport=off  mask{DATA_WIDTH=32, ADDRESS_WIDTH=8, WAIT_STATES_PER_WRITE=0, MAXIMUM_LATENCY=1, SIZE=100, OFFSET=0}
      mask prompts: DATA_WIDTH "Data Width"; ADDRESS_WIDTH "Address Width"; WAIT_STATES_PER_WRITE "Wait States Per Write"; MAXIMUM_LATENCY "Maximum Latency"
      mask help:
      | This is a simulation model of an external RAM block.  It can be used to store and retrieve data from a range of addresses.  It is designed specifically to work with the DSP Builder Video and Image Processing blocks, but may be used for other purposes.
      |
      | As it is a simulation only block, it will not generate HDL when SignalCompiler is run.
      |
      | Parameters
      | =========
      | Data Width - the number of bits used for the data (8,16, 32, 64 or 128 bits only)
      | Address Width - number of bits used for the address (between 1 and 32)
      | Wait States Per Write - choose a fixed number of wait states for each write transfer (between 0 to 10)
      | Maximum Latency - set the latency for pipelined read transfer (between 1 and 255)
      | Size, Offset - to use a range of addresses, choose an offset (start address) and size (number of addresses).  The size added to the offset must be less than 2 ^ address width).
      |
      | Note : If 64 or 128 bits are selected for the data width, the block will attempt to register a Simulink fixed point type of the corresponding width.  This will only work if a valid fixed point license is present on the user's machine.  Please refer to the Simulink help for more information about fixed point licenses.
      mask Help: helpview(fullfile(alt_dspbuilder_get_quartus_rootdir, 'dsp_builder', 'docs', 'ExternalRAM.html'))
      mask Display:
      | port_label('input',1,'WriteData');
      | port_label('input',2,'WriteAddress');
      | port_label('input',3,'ReadAddress');
      | port_label('input',4,'Read');
      | port_label('input',5,'Write');
      | port_label('output',1,'ReadData');
      | port_label('output',2,'WriteWaitRequest');
      | port_label('output',3,'ReadWaitRequest');
      | port_label('output',4,'ReadDataValid');
      | disp('External RAM');
  Extract Bit : S-Function  LoadFcn=alt_dspbuilder_load_block(gcb, 'BlockFactory', 'com.altera.dspbuilder.blockset.iobus.ExtractBit');  FunctionName=sGeneric  Parameters=BusType bwl bwr bitToSelect pipeline_display  EnableBusSupport=off  mask(Extract Bit AlteraBlockset){BusType=Signed Fractional, bwl=8, bwr=1, bitToSelect=0, pipeline_display=0}
      mask prompts: BusType "Bus Type"; bwl "[Number Of Bits].[]"; bwr "[].[Number Of Bits]"; bitToSelect "Select the bit to be extracted from the bus"; pipeline_display "Number Of Pipeline Stages (Calculated)"
      mask help:
      | Reads a Simulink bus in the specified format and outputs the single bit specified.
      | The selected bit is indexed starting from zero for the LSB and increasing to (total bit width - 1) for the MSB.
      mask init:
      | alt_dspbuilder_init('BlockFactory', 'com.altera.dspbuilder.blockset.iobus.ExtractBit', { get_param(gcb, 'BusType') bwl bwr bitToSelect pipeline_display });
      settings: CopyFcn=alt_dspbuilder_add_block(gcb, 'BlockFactory', 'com.altera.dspbuilder.blockset.iobus.ExtractBit');  DeleteFcn=com.altera.dspbuilder.simulation.Mask.delete(gcb);  UndoDeleteFcn=alt_dspbuilder_add_block(gcb, 'BlockFactory', 'com.altera.dspbuilder.blockset.iobus.ExtractBit');  PostSaveFcn=alt_dspbuilder_block_saved(gcb);  NameChangeFcn=alt_dspbuilder_block_renamed(gcb);
      mask Help: helpview(char(com.altera.dspbuilder.simulation.Cache.getBlockTemplate('BlockFactory', 'com.altera.dspbuilder.blockset.iobus.ExtractBit').getHelpFile))
      mask StyleString: popup(Signed Integer|Unsigned Integer|Signed Fractional|Unsigned Fractional),edit,edit,edit,edit
      mask CallbackString: alt_dspbuilder_update_gui('BlockFactory', 'com.altera.dspbuilder.blockset.iobus.ExtractBit', 'BusType', 0);||||
      mask Display:
      | plot([0 0.6 0.6 1 0.6 0.6 0], [0 0 0.25 0.25 0.25 1 1])
      | disp('0')
  FIFO : S-Function  LoadFcn=alt_dspbuilder_load_block(gcb, 'BlockFactory', 'com.altera.dspbuilder.blockset.storage.FIFO');  FunctionName=sGeneric  Parameters=numwords BusType bwl bwr ram_type use_sclr use_les_only showahead_mode allowFloatingPointOverride logOutputs logFile  EnableBusSupport=off  mask(FIFO AlteraBlockset){numwords=64, BusType=Signed Integer, bwl=8, bwr=0, ram_type=AUTO, use_sclr=off, use_les_only=off, showahead_mode=off, allowFloatingPointOverride=on, logOutputs=off, logFile=D:\\allblocks%5Falteradspbuilder2_FIFO%3A%3Aq.fixedpointlog,D:\\allblocks%5Falteradspbuilder2_FIFO%3A%3Afull.fixedpointlog,D:\\allblocks%5Falteradspbuilder2_FIFO%3A%3Aempty.fixedpointlog,D:\\allblocks%5Falteradspbuilder2_FIFO%3A%3Ausedw.fixedpointlog,}
      mask prompts: numwords "Number Of Words In FIFO"; BusType "Data Type"; bwl "[Number Of Bits].[]"; bwr "[].[Number Of Bits]"; ram_type "Memory block type"; use_sclr "Use Synchronous Clear Port (sclr)"; use_les_only "Implement FIFO With Logic Cells Only"; showahead_mode "Use Show-Ahead Mode Of Read Request"; allowFloatingPointOverride "Allow Floating Point Override For This Block"
      mask help:
      | Implements a parameterized, single-clock FIFO buffer.
      |
      | Note that reading an empty FIFO may give unknown (X) in hardware.
      mask init:
      | alt_dspbuilder_init('BlockFactory', 'com.altera.dspbuilder.blockset.storage.FIFO', { numwords get_param(gcb, 'BusType') bwl bwr ram_type use_sclr use_les_only showahead_mode allowFloatingPointOverride logOutputs logFile });
      settings: CopyFcn=alt_dspbuilder_add_block(gcb, 'BlockFactory', 'com.altera.dspbuilder.blockset.storage.FIFO');  DeleteFcn=com.altera.dspbuilder.simulation.Mask.delete(gcb);  UndoDeleteFcn=alt_dspbuilder_add_block(gcb, 'BlockFactory', 'com.altera.dspbuilder.blockset.storage.FIFO');  PostSaveFcn=alt_dspbuilder_block_saved(gcb);  NameChangeFcn=alt_dspbuilder_block_renamed(gcb);
      mask Help: helpview(char(com.altera.dspbuilder.simulation.Cache.getBlockTemplate('BlockFactory', 'com.altera.dspbuilder.blockset.storage.FIFO').getHelpFile))
      mask StyleString: edit,popup(Inferred|Signed Integer|Unsigned Integer|Signed Fractional|Unsigned Fractional),edit,edit,popup(AUTO|M9K|M10K|M20K|MLAB|M144K),checkbox,checkbox,checkbox,checkbox,checkbox,edit
      mask CallbackString: |alt_dspbuilder_update_gui('BlockFactory', 'com.altera.dspbuilder.blockset.storage.FIFO', 'BusType', 1);|||||||||
      mask TabNameString: Main,Main,Main,Main,Main,Optional Ports and Settings,Optional Ports and Settings,Optional Ports and Settings,Optional Ports and Settings,Optional Ports and Settings,Optional Ports and Settings
      mask Display:
      | port_label('input', 1, 'd');
      | port_label('input', 2, 'rreq');
      | port_label('input', 3, 'wreq');
      | port_label('output', 1, 'q');
      | port_label('output', 2, 'full');
      | port_label('output', 3, 'empty');
      | port_label('output', 4, 'usdw(5:0)');
      | disp('FIFO');
  Flipflop : S-Function  LoadFcn=alt_dspbuilder_load_block(gcb, 'BlockFactory', 'com.altera.dspbuilder.blockset.gatecontrol.FlipFlop');  FunctionName=sGeneric  Parameters=mode BusType bwl bwr pipeline_display  EnableBusSupport=off  mask(Flipflop AlteraBlockset){mode=DFFE, BusType=Single Bit, bwl=2, bwr=2, pipeline_display=1}
      mask prompts: BusType "Bus Type"; bwl "[Number Of Bits].[]"; bwr "[].[Number Of Bits]"; pipeline_display "Number Of Pipeline Stages (Calculated)"
      mask help:
      | Implements a D-type flipflop with enable (DFFE) or T-type flipflop with enable (TFFE).
      |
      | If the number of bits is set to more than 1, the block behaves as single-bit flipflops for each bit. For example, for a TFFE flipflop with an n-bit signal, the signal is processed using n 1-bit TFFE flipflops.
      |
      | The aclrn port is an active-low asynchronous clear port. When active this sets the output and internal state to 0 for the remainder/duration of the clock cycle.
      | The aprn port is an active-low asynchronous preset port. When active this sets the output and internal state to 1 for the remainder/duration of the clock cycle.
      |
      | Note that when this block is used for non single-bit data types, each bit of the input is treated separately. For example, in a TFFE flipflop with an n-bit signal, the signal is processed using n 1-bit TFFE flipflops.
      mask init:
      | alt_dspbuilder_init('BlockFactory', 'com.altera.dspbuilder.blockset.gatecontrol.FlipFlop', { get_param(gcb, 'mode') get_param(gcb, 'BusType') bwl bwr pipeline_display });
      settings: CopyFcn=alt_dspbuilder_add_block(gcb, 'BlockFactory', 'com.altera.dspbuilder.blockset.gatecontrol.FlipFlop');  DeleteFcn=com.altera.dspbuilder.simulation.Mask.delete(gcb);  UndoDeleteFcn=alt_dspbuilder_add_block(gcb, 'BlockFactory', 'com.altera.dspbuilder.blockset.gatecontrol.FlipFlop');  PostSaveFcn=alt_dspbuilder_block_saved(gcb);  NameChangeFcn=alt_dspbuilder_block_renamed(gcb);
      mask Help: helpview(char(com.altera.dspbuilder.simulation.Cache.getBlockTemplate('BlockFactory', 'com.altera.dspbuilder.blockset.gatecontrol.FlipFlop').getHelpFile))
      mask StyleString: popup(DFFE|TFFE),popup(Signed Integer|Unsigned Integer|Signed Fractional|Unsigned Fractional|Single Bit),edit,edit,edit
      mask CallbackString: alt_dspbuilder_update_gui('BlockFactory', 'com.altera.dspbuilder.blockset.gatecontrol.FlipFlop', 'mode', 0);|alt_dspbuilder_update_gui('BlockFactory', 'com.altera.dspbuilder.blockset.gatecontrol.FlipFlop', 'BusType', 1);|||
      mask Display:
      | port_label('input', 1, 'input');
      | port_label('input', 2, 'ena');
      | port_label('input', 3, 'aprn');
      | port_label('input', 4, 'aclrn');
      | port_label('output', 1, 'q');
